simulink model "neural_30102019"  (R2018b)
settings: Solver=VariableStepAuto  StartTime=0.0  StopTime=10.0  RelTol=1e-3
libraries: neural x206
(part 4 of 5)

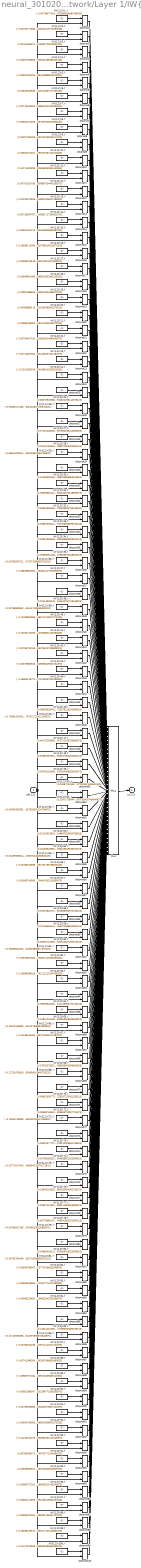
== system neural_30102019/NARX Neural Network/Layer 1/IW{1,2} ==
  "pd{1,2}" : Inport  PortDimensions=10  SampleTime=1
      mask Display: e = 0.06;c1 = [120 230 180]/255;c2 = ([120 230 180]+0)/(256+128);c3 = ([120 230 180]+128)/(256+128);patch([0 1 1 0],[0 0 1 1],c1);patch([0 1 1 1-e 1-e 0+e],[0 0 1 1-e 0+e 0+e],c2);patch([0 0 1 1-e 0+e 0+e],[0 1 1 1-e 1-e 0+e],c3);plot([0 1 1 0 0],[0 0 1 1 0]);
  "IW{1,2}(1,:)'" : Constant  Value=[-0.00798677624919284789850593142546131275594234466552734375;-0.07503946903610680951857148102135397493839263916015625;0.06674643641486444067822958459146320819854736328125;0.049874328743752534276456600537130725570023059844970703125;0.0265489642087564405026345326632508658803999423980712890625;0.013581459089883285429323223070241510868072509765625;0.0285023478571909405498985279336920939385890960693359375;-0.0283260124732715896922474740904362988658249378204345703125;-0.0021890880565128534827878947766066630720160901546478271484375;-0.0190405198631498108474691122182775870896875858306884765625]
      mask Display: e = 0.06;c1 = [120 150 230]/255;c2 = ([120 150 230]+0)/383;c3 = ([120 150 230]+128)/383;patch([0 1 1 0],[0 0 1 1],c1);patch([0 1 1 1-e 1-e 0+e],[0 0 1 1-e 0+e 0+e],c2);patch([0 0 1 1-e 0+e 0+e],[0 1 1 1-e 1-e 0+e],c3);plot([0 1 1 0 0],[0 0 1 1 0]);disp('Weights');
  "IW{1,2}(10,:)'" : Constant  Value=[0.006046723010521692399932280892471680999733507633209228515625;0.061987225392220464403880697545901057310402393341064453125;-0.05670670786149811792853370207012630999088287353515625;-0.04254940000158814739084078837549895979464054107666015625;-0.0229325631839031769676484628917023655958473682403564453125;-0.0119859294762603429962410928055760450661182403564453125;-0.024522060071650482460103859239097801037132740020751953125;0.0229149815121166035292166185399764799512922763824462890625;0.0011335620226404640072115359572535453480668365955352783203125;0.01529158681787430064391575257332078763283789157867431640625]
      mask Display: e = 0.06;c1 = [120 150 230]/255;c2 = ([120 150 230]+0)/383;c3 = ([120 150 230]+128)/383;patch([0 1 1 0],[0 0 1 1],c1);patch([0 1 1 1-e 1-e 0+e],[0 0 1 1-e 0+e 0+e],c2);patch([0 0 1 1-e 0+e 0+e],[0 1 1 1-e 1-e 0+e],c3);plot([0 1 1 0 0],[0 0 1 1 0]);disp('Weights');
  "IW{1,2}(100,:)'" : Constant  Value=[-0.2141767990978555580294795390727813355624675750732421875;-0.128247192817492250416222532294341363012790679931640625;-0.396524834829238503886017497279681265354156494140625;0.3360193962545301449296175633207894861698150634765625;-0.14726526146259144578465338781825266778469085693359375;0.259370633440820841375540339868166483938694000244140625;-0.0037662832053176639561520300247821069206111133098602294921875;0.213933770737092021629877081068116240203380584716796875;0.1274296387092574978083803216577507555484771728515625;0.1001974994320343481657431539133540354669094085693359375]
      mask Display: e = 0.06;c1 = [120 150 230]/255;c2 = ([120 150 230]+0)/383;c3 = ([120 150 230]+128)/383;patch([0 1 1 0],[0 0 1 1],c1);patch([0 1 1 1-e 1-e 0+e],[0 0 1 1-e 0+e 0+e],c2);patch([0 0 1 1-e 0+e 0+e],[0 1 1 1-e 1-e 0+e],c3);plot([0 1 1 0 0],[0 0 1 1 0]);disp('Weights');
  "IW{1,2}(11,:)'" : Constant  Value=[0.421713282934833733062163219074136577546596527099609375;-0.259807602882639099295403184441966004669666290283203125;-0.27575785944389252790642785839736461639404296875;-0.507622809805222008350256146513856947422027587890625;-0.366517809471706257351542035394231788814067840576171875;-0.31407420620104453679033440494094975292682647705078125;-0.27804590867977185819626129159587435424327850341796875;0.1700226487380198381327289780529099516570568084716796875;0.01439665602552794680668579729854172910563647747039794921875;-0.29063000749984058135311215664842166006565093994140625]
      mask Display: e = 0.06;c1 = [120 150 230]/255;c2 = ([120 150 230]+0)/383;c3 = ([120 150 230]+128)/383;patch([0 1 1 0],[0 0 1 1],c1);patch([0 1 1 1-e 1-e 0+e],[0 0 1 1-e 0+e 0+e],c2);patch([0 0 1 1-e 0+e 0+e],[0 1 1 1-e 1-e 0+e],c3);plot([0 1 1 0 0],[0 0 1 1 0]);disp('Weights');
  "IW{1,2}(12,:)'" : Constant  Value=[0.007616107951092995591302337032857394660823047161102294921875;0.072611082900980505883126170374453067779541015625;-0.0648315312200906379569431692289072088897228240966796875;-0.048465470835274519767477130471888813190162181854248046875;-0.025819065849659532385640403617799165658652782440185546875;-0.01322418345371845736779814473038641153834760189056396484375;-0.027704240289464894531068495098224957473576068878173828125;0.0273498164796031305312506987093001953326165676116943359375;0.002044885299220683579080048986043038894422352313995361328125;0.0183814053611497628393234293753266683779656887054443359375]
      mask Display: e = 0.06;c1 = [120 150 230]/255;c2 = ([120 150 230]+0)/383;c3 = ([120 150 230]+128)/383;patch([0 1 1 0],[0 0 1 1],c1);patch([0 1 1 1-e 1-e 0+e],[0 0 1 1-e 0+e 0+e],c2);patch([0 0 1 1-e 0+e 0+e],[0 1 1 1-e 1-e 0+e],c3);plot([0 1 1 0 0],[0 0 1 1 0]);disp('Weights');
  "IW{1,2}(13,:)'" : Constant  Value=[-0.0010537055901131326708652924395437366911210119724273681640625;-0.0239240992321591468272590219612538930959999561309814453125;0.0255710545558940662014268951907070004381239414215087890625;0.0194741137923734007608711493730879737995564937591552734375;0.01128805501537038895321085618661527405492961406707763671875;0.006558522094036949023898586119685205630958080291748046875;0.01174088385979915084844638073491296381689608097076416015625;-0.0077679497450684475978732734802179038524627685546875;0.0011445875772253988507387578721363752265460789203643798828125;-0.004942996574598020921575969310879372642375528812408447265625]
      mask Display: e = 0.06;c1 = [120 150 230]/255;c2 = ([120 150 230]+0)/383;c3 = ([120 150 230]+128)/383;patch([0 1 1 0],[0 0 1 1],c1);patch([0 1 1 1-e 1-e 0+e],[0 0 1 1-e 0+e 0+e],c2);patch([0 0 1 1-e 0+e 0+e],[0 1 1 1-e 1-e 0+e],c3);plot([0 1 1 0 0],[0 0 1 1 0]);disp('Weights');
  "IW{1,2}(14,:)'" : Constant  Value=[0.007355647677175658309678407675846756319515407085418701171875;0.07087343205888226027600040879406151361763477325439453125;-0.0634921597831986928017755644759745337069034576416015625;-0.0474884902285650500886049485416151583194732666015625;-0.025332830322819466228878582114703021943569183349609375;-0.01300591691238471743485849430044254404492676258087158203125;-0.0271698679463006353973497652987134642899036407470703125;0.026631749153002683139224160413505160249769687652587890625;0.00190872735472459066630168678102563717402517795562744140625;0.01788489226589433378489246706521953456103801727294921875]
      mask Display: e = 0.06;c1 = [120 150 230]/255;c2 = ([120 150 230]+0)/383;c3 = ([120 150 230]+128)/383;patch([0 1 1 0],[0 0 1 1],c1);patch([0 1 1 1-e 1-e 0+e],[0 0 1 1-e 0+e 0+e],c2);patch([0 0 1 1-e 0+e 0+e],[0 1 1 1-e 1-e 0+e],c3);plot([0 1 1 0 0],[0 0 1 1 0]);disp('Weights');
  "IW{1,2}(15,:)'" : Constant  Value=[-0.00814161173255857802122381627896174904890358448028564453125;-0.075994613132684296630259268567897379398345947265625;0.06753453343498776184627985230690683238208293914794921875;0.05046449069054280422985669929403229616582393646240234375;0.0268793826447808713309139960756510845385491847991943359375;0.013766439113115279402332902236594236455857753753662109375;0.0288593792420822337074781671617529354989528656005859375;-0.028685856450662162997478077386404038406908512115478515625;-0.0022058677687657114903363453350948475417681038379669189453125;-0.01926966050066114544137008124380372464656829833984375]
      mask Display: e = 0.06;c1 = [120 150 230]/255;c2 = ([120 150 230]+0)/383;c3 = ([120 150 230]+128)/383;patch([0 1 1 0],[0 0 1 1],c1);patch([0 1 1 1-e 1-e 0+e],[0 0 1 1-e 0+e 0+e],c2);patch([0 0 1 1-e 0+e 0+e],[0 1 1 1-e 1-e 0+e],c3);plot([0 1 1 0 0],[0 0 1 1 0]);disp('Weights');
  "IW{1,2}(16,:)'" : Constant  Value=[-0.29668115008275630639644759867223910987377166748046875;-0.1429409359042553562257893418063758872449398040771484375;-0.003996746244826050731280275840617832727730274200439453125;0.1368595726162756542887422028798027895390987396240234375;-0.133843639625026378237038215956999920308589935302734375;-0.382580478673099577680005722868372686207294464111328125;-0.63959980856266540616417159981210716068744659423828125;-0.0904466078387958505313548585036187432706356048583984375;-0.01188476076923118858463812586023777839727699756622314453125;0.421520946410732733067305844087968580424785614013671875]
      mask Display: e = 0.06;c1 = [120 150 230]/255;c2 = ([120 150 230]+0)/383;c3 = ([120 150 230]+128)/383;patch([0 1 1 0],[0 0 1 1],c1);patch([0 1 1 1-e 1-e 0+e],[0 0 1 1-e 0+e 0+e],c2);patch([0 0 1 1-e 0+e 0+e],[0 1 1 1-e 1-e 0+e],c3);plot([0 1 1 0 0],[0 0 1 1 0]);disp('Weights');
  "IW{1,2}(17,:)'" : Constant  Value=[-0.0089611951806888960614383421443562838248908519744873046875;-0.080259490925016996332175267525599338114261627197265625;0.0713183404309283008881692467184620909392833709716796875;0.05343656199492992364685761685905163176357746124267578125;0.02883618272078312949613376758861704729497432708740234375;0.01506443241417236567070148112179595045745372772216796875;0.030848081919005641837738806998459040187299251556396484375;-0.0300637610862332128880414217064753756858408451080322265625;-0.00187828771485964540581548032349701315979473292827606201171875;-0.0199686849717214086330496769505771226249635219573974609375]
      mask Display: e = 0.06;c1 = [120 150 230]/255;c2 = ([120 150 230]+0)/383;c3 = ([120 150 230]+128)/383;patch([0 1 1 0],[0 0 1 1],c1);patch([0 1 1 1-e 1-e 0+e],[0 0 1 1-e 0+e 0+e],c2);patch([0 0 1 1-e 0+e 0+e],[0 1 1 1-e 1-e 0+e],c3);plot([0 1 1 0 0],[0 0 1 1 0]);disp('Weights');
  "IW{1,2}(18,:)'" : Constant  Value=[0.00848961486607587891006776459335014806129038333892822265625;0.07767125028041090006869495709906914271414279937744140625;-0.0690349437182005976065823915632790885865688323974609375;-0.051627200903625637684601912269499734975397586822509765625;-0.0276423307452806042705528710712314932607114315032958984375;-0.0142761761840401735224048707095789723098278045654296875;-0.0296519928027474018172870984244582359679043292999267578125;0.029209814683932501522267699556323350407183170318603515625;0.00206227852408806359985060652206811937503516674041748046875;0.0195439959360052158132692312619838048703968524932861328125]
      mask Display: e = 0.06;c1 = [120 150 230]/255;c2 = ([120 150 230]+0)/383;c3 = ([120 150 230]+128)/383;patch([0 1 1 0],[0 0 1 1],c1);patch([0 1 1 1-e 1-e 0+e],[0 0 1 1-e 0+e 0+e],c2);patch([0 0 1 1-e 0+e 0+e],[0 1 1 1-e 1-e 0+e],c3);plot([0 1 1 0 0],[0 0 1 1 0]);disp('Weights');
  "IW{1,2}(19,:)'" : Constant  Value=[0.0085796862633227659322709968137132818810641765594482421875;0.07930105914873393502251275322123547084629535675048828125;-0.0701868817899373442781296716930228285491466522216796875;-0.0524578341906625500445926491011050529778003692626953125;-0.0279347662272163045626971467072507948614656925201416015625;-0.01430608406650272536320134264542502933181822299957275390625;-0.02998821634027049043424995034001767635345458984375;0.0300247568622749316791242790714022703468799591064453125;0.0023842574512983236677265974634565282030962407588958740234375;0.0201306524346432751115809622888264129869639873504638671875]
      mask Display: e = 0.06;c1 = [120 150 230]/255;c2 = ([120 150 230]+0)/383;c3 = ([120 150 230]+128)/383;patch([0 1 1 0],[0 0 1 1],c1);patch([0 1 1 1-e 1-e 0+e],[0 0 1 1-e 0+e 0+e],c2);patch([0 0 1 1-e 0+e 0+e],[0 1 1 1-e 1-e 0+e],c3);plot([0 1 1 0 0],[0 0 1 1 0]);disp('Weights');
  "IW{1,2}(2,:)'" : Constant  Value=[-0.007357745885256144167951841694730319431982934474945068359375;-0.070887480606621477985385126885375939309597015380859375;0.063502940384915607108240465095150284469127655029296875;0.04749634226454813035189772563171572983264923095703125;0.0253367055119268387575193202110312995500862598419189453125;0.01300762238957645956782815943597597652114927768707275390625;0.0271741310243342193420090779909514822065830230712890625;-0.02663758450105276065489334769154083915054798126220703125;-0.001909879321627074542921942423845393932424485683441162109375;-0.01788894417836141281785700130058103241026401519775390625]
      mask Display: e = 0.06;c1 = [120 150 230]/255;c2 = ([120 150 230]+0)/383;c3 = ([120 150 230]+128)/383;patch([0 1 1 0],[0 0 1 1],c1);patch([0 1 1 1-e 1-e 0+e],[0 0 1 1-e 0+e 0+e],c2);patch([0 0 1 1-e 0+e 0+e],[0 1 1 1-e 1-e 0+e],c3);plot([0 1 1 0 0],[0 0 1 1 0]);disp('Weights');
  "IW{1,2}(20,:)'" : Constant  Value=[0.00486889115257779607481847250483042444102466106414794921875;0.053814783214718685255828489744089893065392971038818359375;-0.05040437383040684282686783035387634299695491790771484375;-0.037941123090531068962061311822253628633916378021240234375;-0.0206956196985309155700338834549256716854870319366455078125;-0.01103117006039725823962616146900472813285887241363525390625;-0.02204589041565323259685982293376582674682140350341796875;0.01952046424261948132095056962498347274959087371826171875;0.0004479422599597729479255214801725060169701464474201202392578125;0.012932389808863638258618067311545019038021564483642578125]
      mask Display: e = 0.06;c1 = [120 150 230]/255;c2 = ([120 150 230]+0)/383;c3 = ([120 150 230]+128)/383;patch([0 1 1 0],[0 0 1 1],c1);patch([0 1 1 1-e 1-e 0+e],[0 0 1 1-e 0+e 0+e],c2);patch([0 0 1 1-e 0+e 0+e],[0 1 1 1-e 1-e 0+e],c3);plot([0 1 1 0 0],[0 0 1 1 0]);disp('Weights');
  "IW{1,2}(21,:)'" : Constant  Value=[0.00866763351667522441434954316719085909426212310791015625;0.0782513990823368865701326058115228079259395599365234375;-0.06959131286961850459960032821982167661190032958984375;-0.052074545671010115388543937342546996660530567169189453125;-0.0279930318366197854185184468178704264573752880096435546875;-0.0145387189400555984220009264618056477047502994537353515625;-0.0299946157684723470338017392577967257238924503326416015625;0.0293345517321344957661910513024849933572113513946533203125;0.0019256041878866268605985379025469228508882224559783935546875;0.01957585198270024584576987081163679249584674835205078125]
      mask Display: e = 0.06;c1 = [120 150 230]/255;c2 = ([120 150 230]+0)/383;c3 = ([120 150 230]+128)/383;patch([0 1 1 0],[0 0 1 1],c1);patch([0 1 1 1-e 1-e 0+e],[0 0 1 1-e 0+e 0+e],c2);patch([0 0 1 1-e 0+e 0+e],[0 1 1 1-e 1-e 0+e],c3);plot([0 1 1 0 0],[0 0 1 1 0]);disp('Weights');
  "IW{1,2}(22,:)'" : Constant  Value=[-0.00708497015945106119183538595507343416102230548858642578125;-0.06905513385735366493900500017844024114310741424560546875;0.062100633166464781764748437353773624636232852935791015625;0.046475737701175169613865278961384319700300693511962890625;0.024835895369398175436259634807356633245944976806640625;0.0127901955732843443380719605784179293550550937652587890625;0.026622792341062316567867895855670212768018245697021484375;-0.0258740150793133893980524362632422707974910736083984375;-0.00175537877912571547989184495008885278366506099700927734375;-0.0173574384835007526628469776142082992009818553924560546875]
      mask Display: e = 0.06;c1 = [120 150 230]/255;c2 = ([120 150 230]+0)/383;c3 = ([120 150 230]+128)/383;patch([0 1 1 0],[0 0 1 1],c1);patch([0 1 1 1-e 1-e 0+e],[0 0 1 1-e 0+e 0+e],c2);patch([0 0 1 1-e 0+e 0+e],[0 1 1 1-e 1-e 0+e],c3);plot([0 1 1 0 0],[0 0 1 1 0]);disp('Weights');
  "IW{1,2}(23,:)'" : Constant  Value=[-0.0074483790066924328299169388856171281076967716217041015625;-0.07149358462194989327631589048905880190432071685791015625;0.06396867056060819012319740295424708165228366851806640625;0.0478356987540748679332835990862804464995861053466796875;0.025504621020149088883588461840190575458109378814697265625;0.01308197665947793790486297638153700972907245159149169921875;0.027358797069702144033609414464081055484712123870849609375;-0.0268889540057255758964682712530702701769769191741943359375;-0.0019589140339770125774643272364983204170130193233489990234375;-0.0180632731988428739400287525995736359618604183197021484375]
      mask Display: e = 0.06;c1 = [120 150 230]/255;c2 = ([120 150 230]+0)/383;c3 = ([120 150 230]+128)/383;patch([0 1 1 0],[0 0 1 1],c1);patch([0 1 1 1-e 1-e 0+e],[0 0 1 1-e 0+e 0+e],c2);patch([0 0 1 1-e 0+e 0+e],[0 1 1 1-e 1-e 0+e],c3);plot([0 1 1 0 0],[0 0 1 1 0]);disp('Weights');
  "IW{1,2}(24,:)'" : Constant  Value=[-0.21911639010605588051561198881245218217372894287109375;-0.01243976575982347516913240070834945072419941425323486328125;-0.276747236623042791592297362512908875942230224609375;0.331513151846347275952808786314562894403934478759765625;0.01530829276420064312402846695704283774830400943756103515625;-0.438908061994073506184577126987278461456298828125;-0.256665691825826047800518381336587481200695037841796875;0.1502781112545034936101018274712259881198406219482421875;-0.060289536450497317743302261305871070362627506256103515625;0.43710829934427819498665712671936489641666412353515625]
      mask Display: e = 0.06;c1 = [120 150 230]/255;c2 = ([120 150 230]+0)/383;c3 = ([120 150 230]+128)/383;patch([0 1 1 0],[0 0 1 1],c1);patch([0 1 1 1-e 1-e 0+e],[0 0 1 1-e 0+e 0+e],c2);patch([0 0 1 1-e 0+e 0+e],[0 1 1 1-e 1-e 0+e],c3);plot([0 1 1 0 0],[0 0 1 1 0]);disp('Weights');
  "IW{1,2}(25,:)'" : Constant  Value=[0.6057391656667754364917755083297379314899444580078125;0.254106170497063021951333894321578554809093475341796875;-0.265690881170252690690603003531577996909618377685546875;-0.429186757129940088528741171103320084512233734130859375;-0.3187917527291614927520413402817212045192718505859375;0.0969355372234030621125810966987046413123607635498046875;-0.282662417338566618330020219218567945063114166259765625;0.13774202595325746312227011003415100276470184326171875;-0.0314014927503679375231371295740245841443538665771484375;-0.155522626980701517140914802439510822296142578125]
      mask Display: e = 0.06;c1 = [120 150 230]/255;c2 = ([120 150 230]+0)/383;c3 = ([120 150 230]+128)/383;patch([0 1 1 0],[0 0 1 1],c1);patch([0 1 1 1-e 1-e 0+e],[0 0 1 1-e 0+e 0+e],c2);patch([0 0 1 1-e 0+e 0+e],[0 1 1 1-e 1-e 0+e],c3);plot([0 1 1 0 0],[0 0 1 1 0]);disp('Weights');
  "IW{1,2}(26,:)'" : Constant  Value=[-0.006801714662381373212307611453297795378603041172027587890625;-0.06714051525852171575792226576595567166805267333984375;0.06063991378496670636710774715538718737661838531494140625;0.045413235239481146432449776284556719474494457244873046875;0.024318707141640506785851272297804825939238071441650390625;0.01256986612047581060302992028709923033602535724639892578125;0.026052733747598109947940514530273503623902797698974609375;-0.0250729610539233427335403803226654417812824249267578125;-0.00158832976997171364426375550493730770540423691272735595703125;-0.0167982994126852532013050023351752315647900104522705078125]
      mask Display: e = 0.06;c1 = [120 150 230]/255;c2 = ([120 150 230]+0)/383;c3 = ([120 150 230]+128)/383;patch([0 1 1 0],[0 0 1 1],c1);patch([0 1 1 1-e 1-e 0+e],[0 0 1 1-e 0+e 0+e],c2);patch([0 0 1 1-e 0+e 0+e],[0 1 1 1-e 1-e 0+e],c3);plot([0 1 1 0 0],[0 0 1 1 0]);disp('Weights');
  "IW{1,2}(27,:)'" : Constant  Value=[0.07131128009140497159279448169399984180927276611328125;-0.0021649104732030465501890770241288919351063668727874755859375;0.357824589089750066950301743418094702064990997314453125;0.085457057636947830747686793984030373394489288330078125;0.2253782000391293116603463886349345557391643524169921875;-0.1387275976291638956983121033772476948797702789306640625;-0.1631566888323170705366038646388915367424488067626953125;-0.01104966204846205383993673621034758980385959148406982421875;0.1563081036359025011162060536662465892732143402099609375;0.27629181597915997148362521329545415937900543212890625]
      mask Display: e = 0.06;c1 = [120 150 230]/255;c2 = ([120 150 230]+0)/383;c3 = ([120 150 230]+128)/383;patch([0 1 1 0],[0 0 1 1],c1);patch([0 1 1 1-e 1-e 0+e],[0 0 1 1-e 0+e 0+e],c2);patch([0 0 1 1-e 0+e 0+e],[0 1 1 1-e 1-e 0+e],c3);plot([0 1 1 0 0],[0 0 1 1 0]);disp('Weights');
  "IW{1,2}(28,:)'" : Constant  Value=[0.10542750616784980766116319728098460473120212554931640625;0.00983497914079346606530673824408950167708098888397216796875;0.1352709594469807818928330789276515133678913116455078125;0.419651828406918558922455986248678527772426605224609375;-0.255329452737788453742240335486712865531444549560546875;-0.286151047620699150453305037444806657731533050537109375;0.23033272063401721840847358180326409637928009033203125;0.13463854237295047600042607882642187178134918212890625;0.079277104628094618998801479392568580806255340576171875;-0.13570287260015423402848000478115864098072052001953125]
      mask Display: e = 0.06;c1 = [120 150 230]/255;c2 = ([120 150 230]+0)/383;c3 = ([120 150 230]+128)/383;patch([0 1 1 0],[0 0 1 1],c1);patch([0 1 1 1-e 1-e 0+e],[0 0 1 1-e 0+e 0+e],c2);patch([0 0 1 1-e 0+e 0+e],[0 1 1 1-e 1-e 0+e],c3);plot([0 1 1 0 0],[0 0 1 1 0]);disp('Weights');
  "IW{1,2}(29,:)'" : Constant  Value=[-0.56624376541417753561091785741155035793781280517578125;0.24101456158054113121380623852019198238849639892578125;0.110371363230960917167777779468451626598834991455078125;0.116837946971778905425054517763783223927021026611328125;0.0032340983457502451951792732387502837809734046459197998046875;-0.08506937579697225471075938685316941700875759124755859375;-0.016568341644388896727324578250772901810705661773681640625;0.417247058757125810490862249935162253677845001220703125;0.4221235175928590432903320106561295688152313232421875;-0.046730484977605825369639802602250711061060428619384765625]
      mask Display: e = 0.06;c1 = [120 150 230]/255;c2 = ([120 150 230]+0)/383;c3 = ([120 150 230]+128)/383;patch([0 1 1 0],[0 0 1 1],c1);patch([0 1 1 1-e 1-e 0+e],[0 0 1 1-e 0+e 0+e],c2);patch([0 0 1 1-e 0+e 0+e],[0 1 1 1-e 1-e 0+e],c3);plot([0 1 1 0 0],[0 0 1 1 0]);disp('Weights');
  "IW{1,2}(3,:)'" : Constant  Value=[0.007534909710501822531492077672510276897810399532318115234375;0.07207083989842300031369859425467438995838165283203125;-0.0644135831885673526553404144578962586820125579833984375;-0.048160216158633979699477123403994482941925525665283203125;-0.025666118012424542216276535100405453704297542572021484375;-0.01315445687860261440860210058190205018036067485809326171875;-0.0275362839360003795741160814714021398685872554779052734375;0.027127517144081396416321894093925948254764080047607421875;0.0020041753028468820875540590265018181526102125644683837890625;0.0182282436409296096091470218425456550903618335723876953125]
      mask Display: e = 0.06;c1 = [120 150 230]/255;c2 = ([120 150 230]+0)/383;c3 = ([120 150 230]+128)/383;patch([0 1 1 0],[0 0 1 1],c1);patch([0 1 1 1-e 1-e 0+e],[0 0 1 1-e 0+e 0+e],c2);patch([0 0 1 1-e 0+e 0+e],[0 1 1 1-e 1-e 0+e],c3);plot([0 1 1 0 0],[0 0 1 1 0]);disp('Weights');
  "IW{1,2}(30,:)'" : Constant  Value=[0.242959481634212604017619696605834178626537322998046875;-0.0417741403241910502774913993562222458422183990478515625;0.658235812223002536569538278854452073574066162109375;-0.33141388019204198744915856877923943102359771728515625;0.416733972177876166309573591206572018563747406005859375;-0.085797801298780840273394687756081111729145050048828125;-0.1883367268382012127414526503343950025737285614013671875;0.09436084962322231761699953267452656291425228118896484375;0.1777182592148270068310722535898094065487384796142578125;0.366611824067617053657386350096203386783599853515625]
      mask Display: e = 0.06;c1 = [120 150 230]/255;c2 = ([120 150 230]+0)/383;c3 = ([120 150 230]+128)/383;patch([0 1 1 0],[0 0 1 1],c1);patch([0 1 1 1-e 1-e 0+e],[0 0 1 1-e 0+e 0+e],c2);patch([0 0 1 1-e 0+e 0+e],[0 1 1 1-e 1-e 0+e],c3);plot([0 1 1 0 0],[0 0 1 1 0]);disp('Weights');
  "IW{1,2}(31,:)'" : Constant  Value=[0.00839862424112747772697584736079079448245465755462646484375;0.07731160948217614958810628422725130803883075714111328125;-0.06869771665354824918825471513628144748508930206298828125;-0.051360203720061357868242879476383677683770656585693359375;-0.02744912374357481865683183741566608659923076629638671875;-0.01413725550662080741870507694102343521080911159515380859375;-0.02945715178367015740779066845789202488958835601806640625;0.0291156286548447003348361050711901043541729450225830078125;0.002121742504950652717654602241736938594840466976165771484375;0.01950610736164447300833302278988412581384181976318359375]
      mask Display: e = 0.06;c1 = [120 150 230]/255;c2 = ([120 150 230]+0)/383;c3 = ([120 150 230]+128)/383;patch([0 1 1 0],[0 0 1 1],c1);patch([0 1 1 1-e 1-e 0+e],[0 0 1 1-e 0+e 0+e],c2);patch([0 0 1 1-e 0+e 0+e],[0 1 1 1-e 1-e 0+e],c3);plot([0 1 1 0 0],[0 0 1 1 0]);disp('Weights');
  "IW{1,2}(32,:)'" : Constant  Value=[0.369346364835059171038977865464403294026851654052734375;0.09681434486543329109853317504530423320829868316650390625;0.582344035522904146517930712434463202953338623046875;-0.56086275654786998945411369277280755341053009033203125;0.039131820943061980389021670134752639569342136383056640625;-0.386360337036403489463509686174802482128143310546875;-0.2685299897506923105794385264744050800800323486328125;-0.1252979787581995907430609804578125476837158203125;0.0768068550977881459029816824113368056714534759521484375;0.354604923895247614584746997934416867792606353759765625]
      mask Display: e = 0.06;c1 = [120 150 230]/255;c2 = ([120 150 230]+0)/383;c3 = ([120 150 230]+128)/383;patch([0 1 1 0],[0 0 1 1],c1);patch([0 1 1 1-e 1-e 0+e],[0 0 1 1-e 0+e 0+e],c2);patch([0 0 1 1-e 0+e 0+e],[0 1 1 1-e 1-e 0+e],c3);plot([0 1 1 0 0],[0 0 1 1 0]);disp('Weights');
  "IW{1,2}(33,:)'" : Constant  Value=[0.0085303821461721988927973114869018900208175182342529296875;0.0792581604486289059696701997381751425564289093017578125;-0.07003614384118529712086598237874568440020084381103515625;-0.052315847801904492853086736658951849676668643951416015625;-0.0277763320123694014418536113453228608705103397369384765625;-0.0141483117667682879725621347688502282835543155670166015625;-0.0298255084064666942111898606526665389537811279296875;0.030092315734682129058086275108507834374904632568359375;0.0025184814520494663674099466987854611943475902080535888671875;0.0202188966654386244325980470648573827929794788360595703125]
      mask Display: e = 0.06;c1 = [120 150 230]/255;c2 = ([120 150 230]+0)/383;c3 = ([120 150 230]+128)/383;patch([0 1 1 0],[0 0 1 1],c1);patch([0 1 1 1-e 1-e 0+e],[0 0 1 1-e 0+e 0+e],c2);patch([0 0 1 1-e 0+e 0+e],[0 1 1 1-e 1-e 0+e],c3);plot([0 1 1 0 0],[0 0 1 1 0]);disp('Weights');
  "IW{1,2}(34,:)'" : Constant  Value=[0.20867893848387997213222888603922910988330841064453125;0.2143074769810318913609847868428914807736873626708984375;-0.24355015505442023648896565646282397210597991943359375;-0.132314619513283882046295047985040582716464996337890625;-0.1363921224583313496214742599477176554501056671142578125;-0.03469070119655058570540262508075102232396602630615234375;0.01404042959988481033273277631678865873254835605621337890625;-0.04500329280021771183317724762673606164753437042236328125;-0.0592947686487854397352492696882109157741069793701171875;-0.0259059849739228138798541323239987832494080066680908203125]
      mask Display: e = 0.06;c1 = [120 150 230]/255;c2 = ([120 150 230]+0)/383;c3 = ([120 150 230]+128)/383;patch([0 1 1 0],[0 0 1 1],c1);patch([0 1 1 1-e 1-e 0+e],[0 0 1 1-e 0+e 0+e],c2);patch([0 0 1 1-e 0+e 0+e],[0 1 1 1-e 1-e 0+e],c3);plot([0 1 1 0 0],[0 0 1 1 0]);disp('Weights');
  "IW{1,2}(35,:)'" : Constant  Value=[0.00960661436772869241351724411970280925743281841278076171875;-0.22744418547777522920938508832477964460849761962890625;0.1376400625764244434190430865783127956092357635498046875;0.049973371980813967307977208065494778566062450408935546875;0.53630542600377995032800981789478100836277008056640625;0.133657341437658505611807413515634834766387939453125;-0.0175443175098067942474511227146649616770446300506591796875;-0.139895193403781537000440948759205639362335205078125;-0.22148819212720349813849907150142826139926910400390625;-0.34148234936702082098491928263683803379535675048828125]
      mask Display: e = 0.06;c1 = [120 150 230]/255;c2 = ([120 150 230]+0)/383;c3 = ([120 150 230]+128)/383;patch([0 1 1 0],[0 0 1 1],c1);patch([0 1 1 1-e 1-e 0+e],[0 0 1 1-e 0+e 0+e],c2);patch([0 0 1 1-e 0+e 0+e],[0 1 1 1-e 1-e 0+e],c3);plot([0 1 1 0 0],[0 0 1 1 0]);disp('Weights');
  "IW{1,2}(36,:)'" : Constant  Value=[-0.007635870215056389694041616422737206448800861835479736328125;-0.072742325179648570365742443755152635276317596435546875;0.064933342151428707911264837093767710030078887939453125;0.04853990443110346719723935393631109036505222320556640625;0.0258565423170550034992487553608953021466732025146484375;0.0132414566793657741128331650770633132196962833404541015625;0.0277453705097093945852737562063339282758533954620361328125;-0.027403647958128544981359908661033841781318187713623046875;-0.002054482437872061362238440551664098165929317474365234375;-0.0184183932665478063139818942772762966342270374298095703125]
      mask Display: e = 0.06;c1 = [120 150 230]/255;c2 = ([120 150 230]+0)/383;c3 = ([120 150 230]+128)/383;patch([0 1 1 0],[0 0 1 1],c1);patch([0 1 1 1-e 1-e 0+e],[0 0 1 1-e 0+e 0+e],c2);patch([0 0 1 1-e 0+e 0+e],[0 1 1 1-e 1-e 0+e],c3);plot([0 1 1 0 0],[0 0 1 1 0]);disp('Weights');
  "IW{1,2}(37,:)'" : Constant  Value=[-0.388498550637164152821156903883093036711215972900390625;0.49736943056161198040143744947272352874279022216796875;0.478056688340715962848292974740616045892238616943359375;-0.187262534023833915330925492526148445904254913330078125;-0.5586836521030094093731577231665141880512237548828125;-0.2406663885132401536903756777974194847047328948974609375;-0.084619108831960276884132099439739249646663665771484375;-0.050153435080850440608291052058120840229094028472900390625;0.19755419481900471367907812236808240413665771484375;0.3355238901682671137649549564230255782604217529296875]
      mask Display: e = 0.06;c1 = [120 150 230]/255;c2 = ([120 150 230]+0)/383;c3 = ([120 150 230]+128)/383;patch([0 1 1 0],[0 0 1 1],c1);patch([0 1 1 1-e 1-e 0+e],[0 0 1 1-e 0+e 0+e],c2);patch([0 0 1 1-e 0+e 0+e],[0 1 1 1-e 1-e 0+e],c3);plot([0 1 1 0 0],[0 0 1 1 0]);disp('Weights');
  "IW{1,2}(38,:)'" : Constant  Value=[0.2511490324976339838514149960246868431568145751953125;-0.128348381365441521761994181360932998359203338623046875;0.06819919537138234566508998568679089657962322235107421875;0.12749848841446420610878931256593205034732818603515625;0.363153841185997972029753100287052802741527557373046875;-0.1776700490802503029641457032994367182254791259765625;-0.242976706441258072377564758426160551607608795166015625;0.06730211923017988262518684905444388277828693389892578125;0.044546208769704047358839460457602399401366710662841796875;-0.061490912827307557531053561206135782413184642791748046875]
      mask Display: e = 0.06;c1 = [120 150 230]/255;c2 = ([120 150 230]+0)/383;c3 = ([120 150 230]+128)/383;patch([0 1 1 0],[0 0 1 1],c1);patch([0 1 1 1-e 1-e 0+e],[0 0 1 1-e 0+e 0+e],c2);patch([0 0 1 1-e 0+e 0+e],[0 1 1 1-e 1-e 0+e],c3);plot([0 1 1 0 0],[0 0 1 1 0]);disp('Weights');
  "IW{1,2}(39,:)'" : Constant  Value=[-0.007688396320664891460394674282952109933830797672271728515625;-0.0730906087948191285352805834918399341404438018798828125;0.0652041463789563013886407816244172863662242889404296875;0.048738059175677757306477388965504360385239124298095703125;0.025956715087612984571574514802705380134284496307373046875;0.01328804358375379988943532083567333756946027278900146484375;0.0278552561390369157745539041570737026631832122802734375;-0.027546115541961457839903459898778237402439117431640625;-0.00207929379404799864750064131158069358207285404205322265625;-0.018516053770908987019527813799868454225361347198486328125]
      mask Display: e = 0.06;c1 = [120 150 230]/255;c2 = ([120 150 230]+0)/383;c3 = ([120 150 230]+128)/383;patch([0 1 1 0],[0 0 1 1],c1);patch([0 1 1 1-e 1-e 0+e],[0 0 1 1-e 0+e 0+e],c2);patch([0 0 1 1-e 0+e 0+e],[0 1 1 1-e 1-e 0+e],c3);plot([0 1 1 0 0],[0 0 1 1 0]);disp('Weights');
  "IW{1,2}(4,:)'" : Constant  Value=[-0.00637465993407875138043738871829191339202225208282470703125;-0.06423379959766921387664950771068106405436992645263671875;0.058423277475708003392274036968956352211534976959228515625;0.04380010836220689374176373576119658537209033966064453125;0.0235373589926678346284649734343474847264587879180908203125;0.012240460689749967093664650974460528232157230377197265625;0.02519039216380007661921780481861787848174571990966796875;-0.0238551637414540496084924825481721200048923492431640625;-0.0013312815436777761073094961119522849912755191326141357421875;-0.0159477076986248751666597200937758316285908222198486328125]
      mask Display: e = 0.06;c1 = [120 150 230]/255;c2 = ([120 150 230]+0)/383;c3 = ([120 150 230]+128)/383;patch([0 1 1 0],[0 0 1 1],c1);patch([0 1 1 1-e 1-e 0+e],[0 0 1 1-e 0+e 0+e],c2);patch([0 0 1 1-e 0+e 0+e],[0 1 1 1-e 1-e 0+e],c3);plot([0 1 1 0 0],[0 0 1 1 0]);disp('Weights');
  "IW{1,2}(40,:)'" : Constant  Value=[-0.12408853983882535410021574762140517123043537139892578125;0.020518071422556787009039425129230949096381664276123046875;-0.86297703007523096641051552069257013499736785888671875;0.019005653693307235363452178944498882628977298736572265625;-0.3965235430061124777267878016573376953601837158203125;0.27873528930856605878574328016838990151882171630859375;0.0902666857515350695706501937820576131343841552734375;-0.33053230245538356424361836616299115121364593505859375;-0.256445713082278314853823530938825570046901702880859375;-0.344709948257618414846348287028376944363117218017578125]
      mask Display: e = 0.06;c1 = [120 150 230]/255;c2 = ([120 150 230]+0)/383;c3 = ([120 150 230]+128)/383;patch([0 1 1 0],[0 0 1 1],c1);patch([0 1 1 1-e 1-e 0+e],[0 0 1 1-e 0+e 0+e],c2);patch([0 0 1 1-e 0+e 0+e],[0 1 1 1-e 1-e 0+e],c3);plot([0 1 1 0 0],[0 0 1 1 0]);disp('Weights');
  "IW{1,2}(41,:)'" : Constant  Value=[-0.2302047629316530119591988068350474350154399871826171875;0.152307209577409896628097385473665781319141387939453125;0.464107114461969894048110063522472046315670013427734375;-0.09824756554074232095530305741704069077968597412109375;0.37441855927202472020809409514185972511768341064453125;0.174697502921786151919292251477600075304508209228515625;0.05809565230288650516943249613177613355219364166259765625;-0.131735813145984426153489721400546841323375701904296875;-0.1338508554063977118442352320926147513091564178466796875;-0.11075163766961894362683693771032267250120639801025390625]
      mask Display: e = 0.06;c1 = [120 150 230]/255;c2 = ([120 150 230]+0)/383;c3 = ([120 150 230]+128)/383;patch([0 1 1 0],[0 0 1 1],c1);patch([0 1 1 1-e 1-e 0+e],[0 0 1 1-e 0+e 0+e],c2);patch([0 0 1 1-e 0+e 0+e],[0 1 1 1-e 1-e 0+e],c3);plot([0 1 1 0 0],[0 0 1 1 0]);disp('Weights');
  "IW{1,2}(42,:)'" : Constant  Value=[-0.007667320498589581985460217339323207852430641651153564453125;-0.07295096307572047911182977486532763577997684478759765625;0.0650954509532313263520109103410504758358001708984375;0.048658492071152394109478933614809648133814334869384765625;0.0259164172440822966614337730106853996403515338897705078125;0.01326922610766675079962961802948484546504914760589599609375;0.0278110608413869135613349925506554427556693553924560546875;-0.02748906435609964338251387516720569692552089691162109375;-0.002069467152952960374567847878779502934776246547698974609375;-0.0184769882848117850127067640642053447663784027099609375]
      mask Display: e = 0.06;c1 = [120 150 230]/255;c2 = ([120 150 230]+0)/383;c3 = ([120 150 230]+128)/383;patch([0 1 1 0],[0 0 1 1],c1);patch([0 1 1 1-e 1-e 0+e],[0 0 1 1-e 0+e 0+e],c2);patch([0 0 1 1-e 0+e 0+e],[0 1 1 1-e 1-e 0+e],c3);plot([0 1 1 0 0],[0 0 1 1 0]);disp('Weights');
  "IW{1,2}(43,:)'" : Constant  Value=[-0.00876983503308761090655476522215394652448594570159912109375;-0.07983504610519187583150824139011092483997344970703125;0.07083189357068257752114703862389433197677135467529296875;0.053012995802292663116705995207667001523077487945556640625;0.028429550368470522803132638500756002031266689300537109375;0.0147229004691482867617224883360904641449451446533203125;0.03047162171117608064907500420304131694138050079345703125;-0.0300556306163373108952807655214201076887547969818115234375;-0.00211315403393556866529223725592601113021373748779296875;-0.0200475237310965247183869308855719282291829586029052734375]
      mask Display: e = 0.06;c1 = [120 150 230]/255;c2 = ([120 150 230]+0)/383;c3 = ([120 150 230]+128)/383;patch([0 1 1 0],[0 0 1 1],c1);patch([0 1 1 1-e 1-e 0+e],[0 0 1 1-e 0+e 0+e],c2);patch([0 0 1 1-e 0+e 0+e],[0 1 1 1-e 1-e 0+e],c3);plot([0 1 1 0 0],[0 0 1 1 0]);disp('Weights');
  "IW{1,2}(44,:)'" : Constant  Value=[-0.196831197211260355839357316654059104621410369873046875;0.004755009296519352619825315997559300740249454975128173828125;0.1973106764472241370089733436543610878288745880126953125;0.058391484374167475224215451135023613460361957550048828125;0.10999830257906619002117309946697787381708621978759765625;-0.29651652439407716332908648837474174797534942626953125;-0.0263660679632789739235132486783186323009431362152099609375;-0.00154190656894976295919474917894831378362141549587249755859375;-0.017058502831990986214893979422413394786417484283447265625;-0.181276988635208857747471711263642646372318267822265625]
      mask Display: e = 0.06;c1 = [120 150 230]/255;c2 = ([120 150 230]+0)/383;c3 = ([120 150 230]+128)/383;patch([0 1 1 0],[0 0 1 1],c1);patch([0 1 1 1-e 1-e 0+e],[0 0 1 1-e 0+e 0+e],c2);patch([0 0 1 1-e 0+e 0+e],[0 1 1 1-e 1-e 0+e],c3);plot([0 1 1 0 0],[0 0 1 1 0]);disp('Weights');
  "IW{1,2}(45,:)'" : Constant  Value=[0.06563629442723693807604234962127520702779293060302734375;0.37819706688799514804344426011084578931331634521484375;-0.3109773356045206771369748821598477661609649658203125;0.3830489996725623402795690708444453775882720947265625;0.25807245818522550617757360669202171266078948974609375;-0.0023620568424722009071015094150425284169614315032958984375;0.0164247632519410984019980759285317617468535900115966796875;-0.3175291683973353595860089626512490212917327880859375;-0.1424539759119330117886903508406248874962329864501953125;-0.355712659745710590986078614150756038725376129150390625]
      mask Display: e = 0.06;c1 = [120 150 230]/255;c2 = ([120 150 230]+0)/383;c3 = ([120 150 230]+128)/383;patch([0 1 1 0],[0 0 1 1],c1);patch([0 1 1 1-e 1-e 0+e],[0 0 1 1-e 0+e 0+e],c2);patch([0 0 1 1-e 0+e 0+e],[0 1 1 1-e 1-e 0+e],c3);plot([0 1 1 0 0],[0 0 1 1 0]);disp('Weights');
  "IW{1,2}(46,:)'" : Constant  Value=[-0.7599242403201496021125649349414743483066558837890625;0.311245626707613298744803387307911179959774017333984375;0.4513301182767204267065608291886746883392333984375;-0.349105266224237931194096518083824776113033294677734375;-0.326415196854076439247904772855690680444240570068359375;0.133872720375285247929042498071794398128986358642578125;0.1479321643633239313775362688829773105680942535400390625;0.0690960871733121706483871093951165676116943359375;0.00748656824979148337317891304110162309370934963226318359375;0.05862141364747007477031814914880669675767421722412109375]
      mask Display: e = 0.06;c1 = [120 150 230]/255;c2 = ([120 150 230]+0)/383;c3 = ([120 150 230]+128)/383;patch([0 1 1 0],[0 0 1 1],c1);patch([0 1 1 1-e 1-e 0+e],[0 0 1 1-e 0+e 0+e],c2);patch([0 0 1 1-e 0+e 0+e],[0 1 1 1-e 1-e 0+e],c3);plot([0 1 1 0 0],[0 0 1 1 0]);disp('Weights');
  "IW{1,2}(47,:)'" : Constant  Value=[0.641752566900068988076100140460766851902008056640625;0.46396433157034755456749053337262012064456939697265625;-0.166504348181084782520855469556408934295177459716796875;-0.067997156009429848833036658106721006333827972412109375;-0.34462816799041195992003849823959171772003173828125;-0.09343619402216431224506010266850353218615055084228515625;0.1527530649089583747457510298772831447422504425048828125;0.0204005276144635545876315774194154073484241962432861328125;-0.09926308259501992470319464700878597795963287353515625;-0.11300737519228508387580944827277562581002712249755859375]
      mask Display: e = 0.06;c1 = [120 150 230]/255;c2 = ([120 150 230]+0)/383;c3 = ([120 150 230]+128)/383;patch([0 1 1 0],[0 0 1 1],c1);patch([0 1 1 1-e 1-e 0+e],[0 0 1 1-e 0+e 0+e],c2);patch([0 0 1 1-e 0+e 0+e],[0 1 1 1-e 1-e 0+e],c3);plot([0 1 1 0 0],[0 0 1 1 0]);disp('Weights');
  "IW{1,2}(48,:)'" : Constant  Value=[0.6286915239198034299761275178752839565277099609375;-0.0923094741738320345714186032637371681630611419677734375;-0.525667897135358774818314486765302717685699462890625;-0.34634196476031398059802768329973332583904266357421875;0.2088975012705418798919509981715236790478229522705078125;0.3189078066195403238225480890832841396331787109375;0.3403261213552808417404094143421389162540435791015625;0.094058258439700559438989557747845537960529327392578125;0.25367785023551780998474214356974698603153228759765625;0.6423720397631289547035748910275287926197052001953125]
      mask Display: e = 0.06;c1 = [120 150 230]/255;c2 = ([120 150 230]+0)/383;c3 = ([120 150 230]+128)/383;patch([0 1 1 0],[0 0 1 1],c1);patch([0 1 1 1-e 1-e 0+e],[0 0 1 1-e 0+e 0+e],c2);patch([0 0 1 1-e 0+e 0+e],[0 1 1 1-e 1-e 0+e],c3);plot([0 1 1 0 0],[0 0 1 1 0]);disp('Weights');
  "IW{1,2}(49,:)'" : Constant  Value=[0.00783110948902149793526827892264918773435056209564208984375;0.074031369192252560740286071450100280344486236572265625;-0.06594149006553172431832621214198297820985317230224609375;-0.049279242551752831802414078765650629065930843353271484375;-0.026234103443511729014669953130578505806624889373779296875;-0.0134209267211293122035176139661416527815163135528564453125;-0.0281590194283356277937802047972581931389868259429931640625;0.027927253735328012862471069865932804532349109649658203125;0.0021400920173110689337381273844584939070045948028564453125;0.01877513474526958103805185373857966624200344085693359375]
      mask Display: e = 0.06;c1 = [120 150 230]/255;c2 = ([120 150 230]+0)/383;c3 = ([120 150 230]+128)/383;patch([0 1 1 0],[0 0 1 1],c1);patch([0 1 1 1-e 1-e 0+e],[0 0 1 1-e 0+e 0+e],c2);patch([0 0 1 1-e 0+e 0+e],[0 1 1 1-e 1-e 0+e],c3);plot([0 1 1 0 0],[0 0 1 1 0]);disp('Weights');
  "IW{1,2}(5,:)'" : Constant  Value=[-0.00801233294552941392729916714188220794312655925750732421875;-0.07520162066456871630126812533490010537207126617431640625;0.0668780520356412611082674857243546284735202789306640625;0.049972253706234648351625082796090282499790191650390625;0.026602236481148712476940687565729604102671146392822265625;0.0136099768024475036021225804461209918372333049774169921875;0.02856019843938605029531885293181403540074825286865234375;-0.0283886932248070926465555174900146084837615489959716796875;-0.0021945498145465127705355801168707330361939966678619384765625;-0.019081380097620094515864508366576046682894229888916015625]
      mask Display: e = 0.06;c1 = [120 150 230]/255;c2 = ([120 150 230]+0)/383;c3 = ([120 150 230]+128)/383;patch([0 1 1 0],[0 0 1 1],c1);patch([0 1 1 1-e 1-e 0+e],[0 0 1 1-e 0+e 0+e],c2);patch([0 0 1 1-e 0+e 0+e],[0 1 1 1-e 1-e 0+e],c3);plot([0 1 1 0 0],[0 0 1 1 0]);disp('Weights');
  "IW{1,2}(50,:)'" : Constant  Value=[0.04587112345533893298377137170973583124577999114990234375;0.102495986757728141380852093789144419133663177490234375;-0.1210533897694758553864602390603977255523204803466796875;0.041216737926025238947236317699207575060427188873291015625;-0.00420419844531171905954725076526301563717424869537353515625;0.11742829263354166713373416541799088008701801300048828125;0.06613098545981598019860570047967485152184963226318359375;-0.1053879141218486414910415760459727607667446136474609375;0.0142281809329760818016996637425108929164707660675048828125;0.09545103750455881386205447824977454729378223419189453125]
      mask Display: e = 0.06;c1 = [120 150 230]/255;c2 = ([120 150 230]+0)/383;c3 = ([120 150 230]+128)/383;patch([0 1 1 0],[0 0 1 1],c1);patch([0 1 1 1-e 1-e 0+e],[0 0 1 1-e 0+e 0+e],c2);patch([0 0 1 1-e 0+e 0+e],[0 1 1 1-e 1-e 0+e],c3);plot([0 1 1 0 0],[0 0 1 1 0]);disp('Weights');
  "IW{1,2}(51,:)'" : Constant  Value=[0.2387273994433078971866279971436597406864166259765625;-0.00415256252339484856206386353960624546743929386138916015625;-0.1823895595057546115125290953073999844491481781005859375;-0.2404200634657055191123475879066972993314266204833984375;-0.1758207127865518970555314126613666303455829620361328125;-0.317659663486635379658906686017871834337711334228515625;0.000400297449155439057956462622911431026295758783817291259765625;-0.1092129714237961568557011560187675058841705322265625;-0.315564834936291671585451013015699572861194610595703125;-0.37927367789468202641245397899183444678783416748046875]
      mask Display: e = 0.06;c1 = [120 150 230]/255;c2 = ([120 150 230]+0)/383;c3 = ([120 150 230]+128)/383;patch([0 1 1 0],[0 0 1 1],c1);patch([0 1 1 1-e 1-e 0+e],[0 0 1 1-e 0+e 0+e],c2);patch([0 0 1 1-e 0+e 0+e],[0 1 1 1-e 1-e 0+e],c3);plot([0 1 1 0 0],[0 0 1 1 0]);disp('Weights');
  "IW{1,2}(52,:)'" : Constant  Value=[-0.5456345059190306212570931165828369557857513427734375;0.336580832127757967331405097866081632673740386962890625;0.333552263557535144666843507366138510406017303466796875;-0.3965929917272177362974616698920726776123046875;-0.359121584020160644623587131718522869050502777099609375;0.3317527056262379314688359954743646085262298583984375;0.438933532281830796062394028922426514327526092529296875;0.0847029401898093947664847291889600455760955810546875;-0.3978526081459203833645688064279966056346893310546875;-0.432851432338583475001314582186751067638397216796875]
      mask Display: e = 0.06;c1 = [120 150 230]/255;c2 = ([120 150 230]+0)/383;c3 = ([120 150 230]+128)/383;patch([0 1 1 0],[0 0 1 1],c1);patch([0 1 1 1-e 1-e 0+e],[0 0 1 1-e 0+e 0+e],c2);patch([0 0 1 1-e 0+e 0+e],[0 1 1 1-e 1-e 0+e],c3);plot([0 1 1 0 0],[0 0 1 1 0]);disp('Weights');
  "IW{1,2}(53,:)'" : Constant  Value=[0.02134319543330766288935507191126816906034946441650390625;0.0126647979815222126720453132975308108143508434295654296875;0.434009204142607962761957196562434546649456024169921875;-0.454152935554614833879583102316246367990970611572265625;-0.11463023260690917426440904591800062917172908782958984375;-0.54220475055219352622515316397766582667827606201171875;0.09271785515872597860376203016130602918565273284912109375;0.04839962870916179882296859204870997928082942962646484375;0.304425936867545043895688650081865489482879638671875;0.3205679640209402325723431204096414148807525634765625]
      mask Display: e = 0.06;c1 = [120 150 230]/255;c2 = ([120 150 230]+0)/383;c3 = ([120 150 230]+128)/383;patch([0 1 1 0],[0 0 1 1],c1);patch([0 1 1 1-e 1-e 0+e],[0 0 1 1-e 0+e 0+e],c2);patch([0 0 1 1-e 0+e 0+e],[0 1 1 1-e 1-e 0+e],c3);plot([0 1 1 0 0],[0 0 1 1 0]);disp('Weights');
  "IW{1,2}(54,:)'" : Constant  Value=[0.2315364856389701408989623132583801634609699249267578125;0.0899495282188080835794607992283999919891357421875;0.139386741858552876127674835515790618956089019775390625;-0.029327407228733538835374616837725625373423099517822265625;0.10465403692043129257882583260652609169483184814453125;-0.1450488583513764029309101033504703082144260406494140625;0.1670683283051941636632165000264649279415607452392578125;-0.007904993108840692450645093458660994656383991241455078125;0.0176673944312657205113481495573068968951702117919921875;-0.08430813677339764333762417436446412466466426849365234375]
      mask Display: e = 0.06;c1 = [120 150 230]/255;c2 = ([120 150 230]+0)/383;c3 = ([120 150 230]+128)/383;patch([0 1 1 0],[0 0 1 1],c1);patch([0 1 1 1-e 1-e 0+e],[0 0 1 1-e 0+e 0+e],c2);patch([0 0 1 1-e 0+e 0+e],[0 1 1 1-e 1-e 0+e],c3);plot([0 1 1 0 0],[0 0 1 1 0]);disp('Weights');
  "IW{1,2}(55,:)'" : Constant  Value=[-0.01009305824310610839866786392349240486510097980499267578125;-0.08194646884067431635845224491276894696056842803955078125;0.07308142019900755459449470663457759656012058258056640625;0.054961818994648241332168225881105172447860240936279296875;0.0305027359921078260185378638880138169042766094207763671875;0.0164685100418424414103757413840867229737341403961181640625;0.032293363089086236927816031538895913399755954742431640625;-0.0298910622616588399214077043097859132103621959686279296875;-0.000749285680339964086336956849976331795915029942989349365234375;-0.0195446095230372880735547624908576835878193378448486328125]
      mask Display: e = 0.06;c1 = [120 150 230]/255;c2 = ([120 150 230]+0)/383;c3 = ([120 150 230]+128)/383;patch([0 1 1 0],[0 0 1 1],c1);patch([0 1 1 1-e 1-e 0+e],[0 0 1 1-e 0+e 0+e],c2);patch([0 0 1 1-e 0+e 0+e],[0 1 1 1-e 1-e 0+e],c3);plot([0 1 1 0 0],[0 0 1 1 0]);disp('Weights');
  "IW{1,2}(56,:)'" : Constant  Value=[-0.0079601368860716496811402720368278096430003643035888671875;-0.0748691664087833552709838613736792467534542083740234375;0.06660895165035206344494866925742826424539089202880859375;0.049772253192793165788021525486328755505383014678955078125;0.0264939457435163540355294031769517459906637668609619140625;0.0135524629523389138208155912934671505354344844818115234375;0.02844251497349893631483297440354363061487674713134765625;-0.028259660889887357193561712165319477207958698272705078125;-0.002182492354442170344464013709284699871204793453216552734375;-0.0189969581126583526853313088622599025256931781768798828125]
      mask Display: e = 0.06;c1 = [120 150 230]/255;c2 = ([120 150 230]+0)/383;c3 = ([120 150 230]+128)/383;patch([0 1 1 0],[0 0 1 1],c1);patch([0 1 1 1-e 1-e 0+e],[0 0 1 1-e 0+e 0+e],c2);patch([0 0 1 1-e 0+e 0+e],[0 1 1 1-e 1-e 0+e],c3);plot([0 1 1 0 0],[0 0 1 1 0]);disp('Weights');
  "IW{1,2}(57,:)'" : Constant  Value=[-0.9240574056008024061981132035725750029087066650390625;-0.235051001672422266164375059815938584506511688232421875;0.6786545452033403424962898498051799833774566650390625;-0.1451895390724890766431798283520038239657878875732421875;0.329777047621199581595163863312336616218090057373046875;-0.09084872424370293853002067407942377030849456787109375;-0.00373585280398288678560536624218002543784677982330322265625;-0.07414170693756548524699923063963069580495357513427734375;-0.3373521618354693440977598584140650928020477294921875;-0.281065689804717633304420587592176161706447601318359375]
      mask Display: e = 0.06;c1 = [120 150 230]/255;c2 = ([120 150 230]+0)/383;c3 = ([120 150 230]+128)/383;patch([0 1 1 0],[0 0 1 1],c1);patch([0 1 1 1-e 1-e 0+e],[0 0 1 1-e 0+e 0+e],c2);patch([0 0 1 1-e 0+e 0+e],[0 1 1 1-e 1-e 0+e],c3);plot([0 1 1 0 0],[0 0 1 1 0]);disp('Weights');
  "IW{1,2}(58,:)'" : Constant  Value=[0.0137833472798940710746240512207805295474827289581298828125;0.2606731672821080980639862900716252624988555908203125;0.21684913401635130814071317217894829809665679931640625;0.0570408891891254210548822811688296496868133544921875;0.1754733489816609759426313530639163218438625335693359375;-0.10645921084077192286798663189983926713466644287109375;0.005724025333909694805700762998412756132893264293670654296875;0.11037747686182523831899260358113679103553295135498046875;-0.046107003413617668463597709660461987368762493133544921875;0.28022159360404341743588929602992720901966094970703125]
      mask Display: e = 0.06;c1 = [120 150 230]/255;c2 = ([120 150 230]+0)/383;c3 = ([120 150 230]+128)/383;patch([0 1 1 0],[0 0 1 1],c1);patch([0 1 1 1-e 1-e 0+e],[0 0 1 1-e 0+e 0+e],c2);patch([0 0 1 1-e 0+e 0+e],[0 1 1 1-e 1-e 0+e],c3);plot([0 1 1 0 0],[0 0 1 1 0]);disp('Weights');
  "IW{1,2}(59,:)'" : Constant  Value=[0.1374566444496357620064230786738335154950618743896484375;-0.1157220185115146182663892204800504259765148162841796875;0.26372810911738231443024460531887598335742950439453125;-0.3368392831515214513871114831999875605106353759765625;0.13819687465548025073758253711275756359100341796875;-0.241125396208886566551399255331489257514476776123046875;-0.04557436446352140790860829611119697801768779754638671875;-0.00914631971451421686702953905978574766777455806732177734375;0.02513869109511490673725120359449647367000579833984375;0.07582269576512164210857491752904024906456470489501953125]
      mask Display: e = 0.06;c1 = [120 150 230]/255;c2 = ([120 150 230]+0)/383;c3 = ([120 150 230]+128)/383;patch([0 1 1 0],[0 0 1 1],c1);patch([0 1 1 1-e 1-e 0+e],[0 0 1 1-e 0+e 0+e],c2);patch([0 0 1 1-e 0+e 0+e],[0 1 1 1-e 1-e 0+e],c3);plot([0 1 1 0 0],[0 0 1 1 0]);disp('Weights');
  "IW{1,2}(6,:)'" : Constant  Value=[0.006450335888016626127716701688541434123180806636810302734375;0.0647505012906349486367929557673051021993160247802734375;-0.058817527542587122457717896395479328930377960205078125;-0.044087152705087902238023644940767553634941577911376953125;-0.0236762154347815341470795402756266412325203418731689453125;-0.01229887531518985936684895676762607763521373271942138671875;-0.025343735586211620092189633624002453871071338653564453125;0.0240716102107036040991250303022752632386982440948486328125;0.00137699656764471932944571275214684646925888955593109130859375;0.016098858234747492890193143466603942215442657470703125]
      mask Display: e = 0.06;c1 = [120 150 230]/255;c2 = ([120 150 230]+0)/383;c3 = ([120 150 230]+128)/383;patch([0 1 1 0],[0 0 1 1],c1);patch([0 1 1 1-e 1-e 0+e],[0 0 1 1-e 0+e 0+e],c2);patch([0 0 1 1-e 0+e 0+e],[0 1 1 1-e 1-e 0+e],c3);plot([0 1 1 0 0],[0 0 1 1 0]);disp('Weights');
  "IW{1,2}(60,:)'" : Constant  Value=[0.0055471269580359694462146080695674754679203033447265625;0.05854176590173883198975346431325306184589862823486328125;-0.05406284868909605467734991179895587265491485595703125;-0.0406195954027717409662301406569895334541797637939453125;-0.0219983393492985922212934468689127243123948574066162109375;-0.01159058496105492240546563920133849023841321468353271484375;-0.0234885040822550884842545571018490591086447238922119140625;0.0214779415191480756164299492638747324235737323760986328125;0.00083659667252587721630874284528545103967189788818359375;0.01429071273310309093951264713950877194292843341827392578125]
      mask Display: e = 0.06;c1 = [120 150 230]/255;c2 = ([120 150 230]+0)/383;c3 = ([120 150 230]+128)/383;patch([0 1 1 0],[0 0 1 1],c1);patch([0 1 1 1-e 1-e 0+e],[0 0 1 1-e 0+e 0+e],c2);patch([0 0 1 1-e 0+e 0+e],[0 1 1 1-e 1-e 0+e],c3);plot([0 1 1 0 0],[0 0 1 1 0]);disp('Weights');
  "IW{1,2}(61,:)'" : Constant  Value=[-0.53606944945962109461135014498722739517688751220703125;-0.0830241725110067718684803139694849960505962371826171875;-0.75443150032839145779917089384980499744415283203125;0.340095781232454374976015287757036276161670684814453125;0.30872404606029579809955976088531315326690673828125;0.285744889265579893322666293897782452404499053955078125;0.360099206842040608922417277426575310528278350830078125;-0.2026811064786902816248215231098583899438381195068359375;0.0750453315907615159385812830805662088096141815185546875;0.151791039693124851783778694880311377346515655517578125]
      mask Display: e = 0.06;c1 = [120 150 230]/255;c2 = ([120 150 230]+0)/383;c3 = ([120 150 230]+128)/383;patch([0 1 1 0],[0 0 1 1],c1);patch([0 1 1 1-e 1-e 0+e],[0 0 1 1-e 0+e 0+e],c2);patch([0 0 1 1-e 0+e 0+e],[0 1 1 1-e 1-e 0+e],c3);plot([0 1 1 0 0],[0 0 1 1 0]);disp('Weights');
  "IW{1,2}(62,:)'" : Constant  Value=[-0.00619601002820189920849980325101569178514182567596435546875;-0.0630114177595981483914755472142132930457592010498046875;0.0574898359684793691659621117651113308966159820556640625;0.043120190958495265010075314648929634131491184234619140625;0.0232085676481234744195081276529890601523220539093017578125;0.01210214818900105272769796016518739634193480014801025390625;0.024827145332792212306660672993530170060694217681884765625;-0.0233433762894651418429159406286999001167714595794677734375;-0.00122342594022647349095989088851865744800306856632232666015625;-0.01559044695096782097432086544586127274669706821441650390625]
      mask Display: e = 0.06;c1 = [120 150 230]/255;c2 = ([120 150 230]+0)/383;c3 = ([120 150 230]+128)/383;patch([0 1 1 0],[0 0 1 1],c1);patch([0 1 1 1-e 1-e 0+e],[0 0 1 1-e 0+e 0+e],c2);patch([0 0 1 1-e 0+e 0+e],[0 1 1 1-e 1-e 0+e],c3);plot([0 1 1 0 0],[0 0 1 1 0]);disp('Weights');
  "IW{1,2}(63,:)'" : Constant  Value=[-0.10899598156518598701669731099173077382147312164306640625;-0.38338791758090084993426671644556336104869842529296875;0.0946649833586936384488552675975370220839977264404296875;0.09731050329213837557507105202603270299732685089111328125;-0.054359892437083716376644559886699425987899303436279296875;-0.35367633474813320315632836354780010879039764404296875;-0.31759021228900718991638996158144436776638031005859375;-0.359423220623583394850442118695355020463466644287109375;0.039583397966895271513632081905598170123994350433349609375;-0.03578591740633675633009858074728981591761112213134765625]
      mask Display: e = 0.06;c1 = [120 150 230]/255;c2 = ([120 150 230]+0)/383;c3 = ([120 150 230]+128)/383;patch([0 1 1 0],[0 0 1 1],c1);patch([0 1 1 1-e 1-e 0+e],[0 0 1 1-e 0+e 0+e],c2);patch([0 0 1 1-e 0+e 0+e],[0 1 1 1-e 1-e 0+e],c3);plot([0 1 1 0 0],[0 0 1 1 0]);disp('Weights');
  "IW{1,2}(64,:)'" : Constant  Value=[0.03538323284052395656384959465867723338305950164794921875;-0.0234334058790095674240649969988226075656712055206298828125;-0.42643364114070114734289518310106359422206878662109375;-0.1154642896338170798831157526365132071077823638916015625;0.0734347540454273473020663232091465033590793609619140625;0.1432105764030799921471270863548852503299713134765625;0.2373997394507786073969413109807646833360195159912109375;-0.1340305425873167255446105627925135195255279541015625;0.14757511966163694427933705810573883354663848876953125;0.166998434214602031744334453833289444446563720703125]
      mask Display: e = 0.06;c1 = [120 150 230]/255;c2 = ([120 150 230]+0)/383;c3 = ([120 150 230]+128)/383;patch([0 1 1 0],[0 0 1 1],c1);patch([0 1 1 1-e 1-e 0+e],[0 0 1 1-e 0+e 0+e],c2);patch([0 0 1 1-e 0+e 0+e],[0 1 1 1-e 1-e 0+e],c3);plot([0 1 1 0 0],[0 0 1 1 0]);disp('Weights');
  "IW{1,2}(65,:)'" : Constant  Value=[0.10841242199356089515038803483548690564930438995361328125;0.0675547742727371780535605694240075536072254180908203125;0.137038573566636900924464725903817452490329742431640625;0.36468071405031532439267039080732502043247222900390625;0.366486629144569475702297722818912006914615631103515625;0.337861284676247375369229075658950023353099822998046875;-0.1189152256869487056523126966567360796034336090087890625;-0.137988181002448861978137983896885998547077178955078125;-0.12120846820254037312647454882608144544064998626708984375;-0.366735535715038973858526105686905793845653533935546875]
      mask Display: e = 0.06;c1 = [120 150 230]/255;c2 = ([120 150 230]+0)/383;c3 = ([120 150 230]+128)/383;patch([0 1 1 0],[0 0 1 1],c1);patch([0 1 1 1-e 1-e 0+e],[0 0 1 1-e 0+e 0+e],c2);patch([0 0 1 1-e 0+e 0+e],[0 1 1 1-e 1-e 0+e],c3);plot([0 1 1 0 0],[0 0 1 1 0]);disp('Weights');
  "IW{1,2}(66,:)'" : Constant  Value=[-0.348734486931703113743452604467165656387805938720703125;0.268744041330844563031376992512377910315990447998046875;0.1742988603789233092999921836963039822876453399658203125;-0.2306781715802361520939456340784090571105480194091796875;-0.2006065768255071990466831266530789434909820556640625;0.11314863663363418366802903847201378084719181060791015625;-0.257625635827576082714784888594294898211956024169921875;-0.237921603946771309523455784074030816555023193359375;-0.063236469011119178507129845456802286207675933837890625;-0.11474434283012026336567856787951313890516757965087890625]
      mask Display: e = 0.06;c1 = [120 150 230]/255;c2 = ([120 150 230]+0)/383;c3 = ([120 150 230]+128)/383;patch([0 1 1 0],[0 0 1 1],c1);patch([0 1 1 1-e 1-e 0+e],[0 0 1 1-e 0+e 0+e],c2);patch([0 0 1 1-e 0+e 0+e],[0 1 1 1-e 1-e 0+e],c3);plot([0 1 1 0 0],[0 0 1 1 0]);disp('Weights');
  "IW{1,2}(67,:)'" : Constant  Value=[-0.1413634945235867912405325341751449741423130035400390625;-0.17718575184882301432054418910411186516284942626953125;0.1392756329402569936970479602678096853196620941162109375;-0.005290470883346384996237521392004055087454617023468017578125;0.40228142354877782782551776108448393642902374267578125;0.354869022084309426734449743889854289591312408447265625;-0.0688696189066963782021701945268432609736919403076171875;0.022461421504704405516239518192378454841673374176025390625;-0.11409576252366725179765438724643900059163570404052734375;0.184000856085178854382178315063356421887874603271484375]
      mask Display: e = 0.06;c1 = [120 150 230]/255;c2 = ([120 150 230]+0)/383;c3 = ([120 150 230]+128)/383;patch([0 1 1 0],[0 0 1 1],c1);patch([0 1 1 1-e 1-e 0+e],[0 0 1 1-e 0+e 0+e],c2);patch([0 0 1 1-e 0+e 0+e],[0 1 1 1-e 1-e 0+e],c3);plot([0 1 1 0 0],[0 0 1 1 0]);disp('Weights');
  "IW{1,2}(68,:)'" : Constant  Value=[0.0700257505156910708965511958012939430773258209228515625;-0.293881051126017478480889622005634009838104248046875;-0.2131614825356262787892092092079110443592071533203125;0.5642235713089573945211441241553984582424163818359375;0.1630483113949482143478775242328993044793605804443359375;0.6689435152123888173036903026513755321502685546875;-0.127419347508939628799140564296976663172245025634765625;0.09368561333392581846890578844977426342666149139404296875;0.039210251806375939764848226332105696201324462890625;0.07418570426289795849417174622431048192083835601806640625]
      mask Display: e = 0.06;c1 = [120 150 230]/255;c2 = ([120 150 230]+0)/383;c3 = ([120 150 230]+128)/383;patch([0 1 1 0],[0 0 1 1],c1);patch([0 1 1 1-e 1-e 0+e],[0 0 1 1-e 0+e 0+e],c2);patch([0 0 1 1-e 0+e 0+e],[0 1 1 1-e 1-e 0+e],c3);plot([0 1 1 0 0],[0 0 1 1 0]);disp('Weights');
  "IW{1,2}(69,:)'" : Constant  Value=[-0.17225478928316173554691204117261804640293121337890625;0.04136361889152286031023919576909975148737430572509765625;-0.06792813701780235635663274251783150248229503631591796875;0.6373322164630554897968295335886068642139434814453125;-0.217858633751632335684433883216115646064281463623046875;0.2184348251170423471645420931963599286973476409912109375;0.23289858629858162242243224682169966399669647216796875;0.37898954404875995205514982444583438336849212646484375;0.1490379247013667585175511476336396299302577972412109375;-0.293229068949460380810734250189852900803089141845703125]
      mask Display: e = 0.06;c1 = [120 150 230]/255;c2 = ([120 150 230]+0)/383;c3 = ([120 150 230]+128)/383;patch([0 1 1 0],[0 0 1 1],c1);patch([0 1 1 1-e 1-e 0+e],[0 0 1 1-e 0+e 0+e],c2);patch([0 0 1 1-e 0+e 0+e],[0 1 1 1-e 1-e 0+e],c3);plot([0 1 1 0 0],[0 0 1 1 0]);disp('Weights');
  "IW{1,2}(7,:)'" : Constant  Value=[-0.00779042800484481927358881847567317890934646129608154296875;-0.073764247797119264493659329673391766846179962158203125;0.06573108488620944822589109435284626670181751251220703125;0.049124517432346616330196553690257132984697818756103515625;0.026154124205801564106987910918178386054933071136474609375;0.01338193915615334093904831291865775710903108119964599609375;0.028071529149404424174907290989722241647541522979736328125;-0.0278196942790493555175412865310136112384498119354248046875;-0.002123941912192028359795958891709233284927904605865478515625;-0.0187024151279206220233053414858659380115568637847900390625]
      mask Display: e = 0.06;c1 = [120 150 230]/255;c2 = ([120 150 230]+0)/383;c3 = ([120 150 230]+128)/383;patch([0 1 1 0],[0 0 1 1],c1);patch([0 1 1 1-e 1-e 0+e],[0 0 1 1-e 0+e 0+e],c2);patch([0 0 1 1-e 0+e 0+e],[0 1 1 1-e 1-e 0+e],c3);plot([0 1 1 0 0],[0 0 1 1 0]);disp('Weights');
  "IW{1,2}(70,:)'" : Constant  Value=[0.00661505773533277267872687588123881141655147075653076171875;0.06587283751865082026544229165665456093847751617431640625;-0.059673448014316975152038224905481911264359951019287109375;-0.04471010675747062734775028047806699760258197784423828125;-0.023977774381534151804107324323922512121498584747314453125;-0.0124258578937376830408911843051100731827318668365478515625;-0.025676619354611192325155144544623908586800098419189453125;0.02454186821815675101365883392645628191530704498291015625;0.0014763640377913737379567127305790563696064054965972900390625;0.0164273241383162856010802244099977542646229267120361328125]
      mask Display: e = 0.06;c1 = [120 150 230]/255;c2 = ([120 150 230]+0)/383;c3 = ([120 150 230]+128)/383;patch([0 1 1 0],[0 0 1 1],c1);patch([0 1 1 1-e 1-e 0+e],[0 0 1 1-e 0+e 0+e],c2);patch([0 0 1 1-e 0+e 0+e],[0 1 1 1-e 1-e 0+e],c3);plot([0 1 1 0 0],[0 0 1 1 0]);disp('Weights');
  "IW{1,2}(71,:)'" : Constant  Value=[0.00856734842360248709247638743136121775023639202117919921875;0.0805211552355509507794550927428645081818103790283203125;-0.0707358759247143920045886034131399355828762054443359375;-0.052802839899786492561251094457475119270384311676025390625;-0.027846523517490680277308712220474262721836566925048828125;-0.01398500447484574658874034724931334494613111019134521484375;-0.0298661384514750764818113992760117980651557445526123046875;0.0308240321198023324578141313168089254759252071380615234375;0.0029266314388043369008884919679758240818046033382415771484375;0.0207754090007528924299862183033837936818599700927734375]
      mask Display: e = 0.06;c1 = [120 150 230]/255;c2 = ([120 150 230]+0)/383;c3 = ([120 150 230]+128)/383;patch([0 1 1 0],[0 0 1 1],c1);patch([0 1 1 1-e 1-e 0+e],[0 0 1 1-e 0+e 0+e],c2);patch([0 0 1 1-e 0+e 0+e],[0 1 1 1-e 1-e 0+e],c3);plot([0 1 1 0 0],[0 0 1 1 0]);disp('Weights');
  "IW{1,2}(72,:)'" : Constant  Value=[-0.10949718999100023497650369108669110573828220367431640625;-0.2941903442223254838694401769316755235195159912109375;-0.207423660958987898794703141902573406696319580078125;-0.1801758309294279047918507785652764141559600830078125;-0.299656438307677797094896732232882641255855560302734375;-0.1024800888478863691855025308541371487081050872802734375;0.2212918490883914734990156603089417330920696258544921875;0.0981645332169653606069203988226945511996746063232421875;0.092067304055237830784363950442639179527759552001953125;-0.1471544847929217303406090877615497447550296783447265625]
      mask Display: e = 0.06;c1 = [120 150 230]/255;c2 = ([120 150 230]+0)/383;c3 = ([120 150 230]+128)/383;patch([0 1 1 0],[0 0 1 1],c1);patch([0 1 1 1-e 1-e 0+e],[0 0 1 1-e 0+e 0+e],c2);patch([0 0 1 1-e 0+e 0+e],[0 1 1 1-e 1-e 0+e],c3);plot([0 1 1 0 0],[0 0 1 1 0]);disp('Weights');
  "IW{1,2}(73,:)'" : Constant  Value=[0.00619377737609348721914415136780007742345333099365234375;0.0629961186040937926033933536018594168126583099365234375;-0.057478145294033979040282389405547291971743106842041015625;-0.043111672615652428530719220134415081702172756195068359375;-0.02320444882004812914289004766033031046390533447265625;-0.012100414925658477260927980978522100485861301422119140625;-0.0248225935625863251832168288046887028031051158905029296875;0.0233369738982593007137200658007714082486927509307861328125;0.00122207966707225880627352143648067794856615364551544189453125;0.0155859790920187570029131762794349924661219120025634765625]
      mask Display: e = 0.06;c1 = [120 150 230]/255;c2 = ([120 150 230]+0)/383;c3 = ([120 150 230]+128)/383;patch([0 1 1 0],[0 0 1 1],c1);patch([0 1 1 1-e 1-e 0+e],[0 0 1 1-e 0+e 0+e],c2);patch([0 0 1 1-e 0+e 0+e],[0 1 1 1-e 1-e 0+e],c3);plot([0 1 1 0 0],[0 0 1 1 0]);disp('Weights');
  "IW{1,2}(74,:)'" : Constant  Value=[0.00796283251811428192945552240189499570988118648529052734375;0.074886451927383468341048455840791575610637664794921875;-0.0666228745686030798811572140039061196148395538330078125;-0.049782581071489868940194156721190665848553180694580078125;-0.0264994907925405580317868015072235721163451671600341796875;-0.01355536574916115476197031597394015989266335964202880859375;-0.028448548854529513707500854025056469254195690155029296875;0.0282664173157827249005524805625100270844995975494384765625;0.0021831979728401339733989683367099132738076150417327880859375;0.0190014068617429289498321764995125704444944858551025390625]
      mask Display: e = 0.06;c1 = [120 150 230]/255;c2 = ([120 150 230]+0)/383;c3 = ([120 150 230]+128)/383;patch([0 1 1 0],[0 0 1 1],c1);patch([0 1 1 1-e 1-e 0+e],[0 0 1 1-e 0+e 0+e],c2);patch([0 0 1 1-e 0+e 0+e],[0 1 1 1-e 1-e 0+e],c3);plot([0 1 1 0 0],[0 0 1 1 0]);disp('Weights');
  "IW{1,2}(75,:)'" : Constant  Value=[-0.307734176432365946762814701287425123155117034912109375;-0.1286169436302920521253412289297557435929775238037109375;0.0128343455476772443091260100800354848615825176239013671875;0.238880027745760725732537821386358700692653656005859375;-0.324733369235029101229628167857299558818340301513671875;-0.043018970852601430554518202598046627826988697052001953125;-0.3787219238720374026030413006083108484745025634765625;-0.194347652908113233127807006894727237522602081298828125;-0.20620012345346150350877678647520951926708221435546875;0.26268888807607027047197334468364715576171875]
      mask Display: e = 0.06;c1 = [120 150 230]/255;c2 = ([120 150 230]+0)/383;c3 = ([120 150 230]+128)/383;patch([0 1 1 0],[0 0 1 1],c1);patch([0 1 1 1-e 1-e 0+e],[0 0 1 1-e 0+e 0+e],c2);patch([0 0 1 1-e 0+e 0+e],[0 1 1 1-e 1-e 0+e],c3);plot([0 1 1 0 0],[0 0 1 1 0]);disp('Weights');
  "IW{1,2}(76,:)'" : Constant  Value=[0.13849101833063082178654212839319370687007904052734375;-0.05314914385130535545709307143624755553901195526123046875;0.497122642672203018943122287964797578752040863037109375;0.4110924394139150450655506574548780918121337890625;0.2290434115684903126908267267936025746166706085205078125;0.06872317245472493729696594755296246148645877838134765625;0.1508650196702952805960507021154626272618770599365234375;-0.03926928713022224959328099203048623166978359222412109375;0.04652758211313645642093206333811394870281219482421875;-0.032724594777101066733759893168098642490804195404052734375]
      mask Display: e = 0.06;c1 = [120 150 230]/255;c2 = ([120 150 230]+0)/383;c3 = ([120 150 230]+128)/383;patch([0 1 1 0],[0 0 1 1],c1);patch([0 1 1 1-e 1-e 0+e],[0 0 1 1-e 0+e 0+e],c2);patch([0 0 1 1-e 0+e 0+e],[0 1 1 1-e 1-e 0+e],c3);plot([0 1 1 0 0],[0 0 1 1 0]);disp('Weights');
  "IW{1,2}(77,:)'" : Constant  Value=[0.005574113616244929549081721376069253892637789249420166015625;0.058728606689789540629131892046643770299851894378662109375;-0.05420665289295367728072960744611918926239013671875;-0.040724680326161950827401625474522006697952747344970703125;-0.0220492819712536126941504477372291148640215396881103515625;-0.01161224825351592215838536503724753856658935546875;-0.0235448929700899332873031966073540388606488704681396484375;0.0215556748283516376452073615155313746072351932525634765625;0.000852442945711465106979620731664226696011610329151153564453125;0.0143447791513248400219193712246124050579965114593505859375]
      mask Display: e = 0.06;c1 = [120 150 230]/255;c2 = ([120 150 230]+0)/383;c3 = ([120 150 230]+128)/383;patch([0 1 1 0],[0 0 1 1],c1);patch([0 1 1 1-e 1-e 0+e],[0 0 1 1-e 0+e 0+e],c2);patch([0 0 1 1-e 0+e 0+e],[0 1 1 1-e 1-e 0+e],c3);plot([0 1 1 0 0],[0 0 1 1 0]);disp('Weights');
  "IW{1,2}(78,:)'" : Constant  Value=[0.00778986147982392573840826344166998751461505889892578125;0.07376052036204695794285868259976268745958805084228515625;-0.06572815645568723386116261053757625631988048553466796875;-0.049122366099054660948386441532420576550066471099853515625;-0.0261530169622286035036040630075149238109588623046875;-0.01338140417814025033560465516302429023198783397674560546875;-0.028070317282863473107301643949540448375046253204345703125;0.027818188533738776035963979893494979478418827056884765625;0.002123708470767689780733800120060550398193299770355224609375;0.0187013942688763375177263270643379655666649341583251953125]
      mask Display: e = 0.06;c1 = [120 150 230]/255;c2 = ([120 150 230]+0)/383;c3 = ([120 150 230]+128)/383;patch([0 1 1 0],[0 0 1 1],c1);patch([0 1 1 1-e 1-e 0+e],[0 0 1 1-e 0+e 0+e],c2);patch([0 0 1 1-e 0+e 0+e],[0 1 1 1-e 1-e 0+e],c3);plot([0 1 1 0 0],[0 0 1 1 0]);disp('Weights');
  "IW{1,2}(79,:)'" : Constant  Value=[-0.007669272951113287502267201745098645915277302265167236328125;-0.07296390571697948523866017467298661358654499053955078125;0.0651055183839352180630299926633597351610660552978515625;0.048665859773598545146011673523389617912471294403076171875;0.0259201444044292912682880825059328344650566577911376953125;0.0132709621382449578785855948126481962390244007110595703125;0.0278151490549122422379912933365631033666431903839111328125;-0.0274943561290978688571584598321351222693920135498046875;-0.0020703849502057354754758211612397644785232841968536376953125;-0.0184806142730388443806699427796047530137002468109130859375]
      mask Display: e = 0.06;c1 = [120 150 230]/255;c2 = ([120 150 230]+0)/383;c3 = ([120 150 230]+128)/383;patch([0 1 1 0],[0 0 1 1],c1);patch([0 1 1 1-e 1-e 0+e],[0 0 1 1-e 0+e 0+e],c2);patch([0 0 1 1-e 0+e 0+e],[0 1 1 1-e 1-e 0+e],c3);plot([0 1 1 0 0],[0 0 1 1 0]);disp('Weights');
  "IW{1,2}(8,:)'" : Constant  Value=[-0.008313732556325191536128471625488600693643093109130859375;-0.0769263054143709823495811406246502883732318878173828125;0.068345574737835701473187555166077800095081329345703125;0.051085047184044031498562077331371256150305271148681640625;0.02726221838423707743981339035599376074969768524169921875;0.01400841354140890289425858128424806636758148670196533203125;0.029264535076659027590384454242666834034025669097900390625;-0.0290019931491190853523054471452269353903830051422119140625;-0.0021656411364033623968838870865738499560393393039703369140625;-0.01945110719536731480605595834276755340397357940673828125]
      mask Display: e = 0.06;c1 = [120 150 230]/255;c2 = ([120 150 230]+0)/383;c3 = ([120 150 230]+128)/383;patch([0 1 1 0],[0 0 1 1],c1);patch([0 1 1 1-e 1-e 0+e],[0 0 1 1-e 0+e 0+e],c2);patch([0 0 1 1-e 0+e 0+e],[0 1 1 1-e 1-e 0+e],c3);plot([0 1 1 0 0],[0 0 1 1 0]);disp('Weights');
  "IW{1,2}(80,:)'" : Constant  Value=[0.00866304211342162899800456443699658848345279693603515625;0.07959986419815578972958292069961316883563995361328125;-0.0705283139969269112778960106879821978509426116943359375;-0.052745798028333977514048314105821191333234310150146484375;-0.0281717302729052911092200162102017202414572238922119140625;-0.01449933846294436390333970621213666163384914398193359375;-0.0302255867905414886409598551608723937533795833587646484375;0.0300666835483465212652820497396533028222620487213134765625;0.0022709535248286688395580323884814788470976054668426513671875;0.020111919562960524354711111527649336494505405426025390625]
      mask Display: e = 0.06;c1 = [120 150 230]/255;c2 = ([120 150 230]+0)/383;c3 = ([120 150 230]+128)/383;patch([0 1 1 0],[0 0 1 1],c1);patch([0 1 1 1-e 1-e 0+e],[0 0 1 1-e 0+e 0+e],c2);patch([0 0 1 1-e 0+e 0+e],[0 1 1 1-e 1-e 0+e],c3);plot([0 1 1 0 0],[0 0 1 1 0]);disp('Weights');
  "IW{1,2}(81,:)'" : Constant  Value=[-0.0078378044837576731074246794150894857011735439300537109375;-0.07407522641225740278603240085431025363504886627197265625;0.06597612814385989121745978991384617984294891357421875;0.04930474080098067035660136525621055625379085540771484375;0.02624734420335668449997257312134024687111377716064453125;0.0134274406363567265498826230896156630478799343109130859375;0.028173494976577888315727449253245140425860881805419921875;-0.0279448536556729208724103585836928687058389186859130859375;-0.00214264347637391390499761456567284767515957355499267578125;-0.0187869982061720126875759007134547573514282703399658203125]
      mask Display: e = 0.06;c1 = [120 150 230]/255;c2 = ([120 150 230]+0)/383;c3 = ([120 150 230]+128)/383;patch([0 1 1 0],[0 0 1 1],c1);patch([0 1 1 1-e 1-e 0+e],[0 0 1 1-e 0+e 0+e],c2);patch([0 0 1 1-e 0+e 0+e],[0 1 1 1-e 1-e 0+e],c3);plot([0 1 1 0 0],[0 0 1 1 0]);disp('Weights');
  "IW{1,2}(82,:)'" : Constant  Value=[-0.00849789047607767307479509355516711366362869739532470703125;-0.07770128606153527128785896138651878573000431060791015625;0.0690635081289484309419179908218211494386196136474609375;0.051649989837669836589828520345690776593983173370361328125;0.0276594445658981842595114386540444684214890003204345703125;0.01428874829386965646105256411146910977549850940704345703125;0.0296690258961389875802527882342474185861647129058837890625;-0.0292170343451981680271689612027330440469086170196533203125;-0.002056323516251346884831097128198962309397757053375244140625;-0.0195464462250868990789154366893853875808417797088623046875]
      mask Display: e = 0.06;c1 = [120 150 230]/255;c2 = ([120 150 230]+0)/383;c3 = ([120 150 230]+128)/383;patch([0 1 1 0],[0 0 1 1],c1);patch([0 1 1 1-e 1-e 0+e],[0 0 1 1-e 0+e 0+e],c2);patch([0 0 1 1-e 0+e 0+e],[0 1 1 1-e 1-e 0+e],c3);plot([0 1 1 0 0],[0 0 1 1 0]);disp('Weights');
  "IW{1,2}(83,:)'" : Constant  Value=[-0.00829318650636188918479074771994419279508292675018310546875;-0.07682521247041386447396149605992832221090793609619140625;0.0682549143437376215626244402301381342113018035888671875;0.051014815615542281890260056798069854266941547393798828125;0.027216405744303472091782936104209511540830135345458984375;0.01397784265785556763461716656138378311879932880401611328125;0.029216738173555807656089911006347392685711383819580078125;-0.0289702103828696488907468165052705444395542144775390625;-0.002174048169437101975243198381804177188314497470855712890625;-0.019434400615108649024165288210497237741947174072265625]
      mask Display: e = 0.06;c1 = [120 150 230]/255;c2 = ([120 150 230]+0)/383;c3 = ([120 150 230]+128)/383;patch([0 1 1 0],[0 0 1 1],c1);patch([0 1 1 1-e 1-e 0+e],[0 0 1 1-e 0+e 0+e],c2);patch([0 0 1 1-e 0+e 0+e],[0 1 1 1-e 1-e 0+e],c3);plot([0 1 1 0 0],[0 0 1 1 0]);disp('Weights');
  "IW{1,2}(84,:)'" : Constant  Value=[-0.49368229820591980061550430036731995642185211181640625;-0.45898684946655665672921031728037633001804351806640625;-0.0762255724241505394633833248008158989250659942626953125;-0.05395222340349768719303114039576030336320400238037109375;0.36559230440862855449069002133910544216632843017578125;0.05339374248459594074489587001153267920017242431640625;0.32768687612741675962979570613242685794830322265625;0.2243970173181835392473004731073160655796527862548828125;0.06617409755495211320930337706158752553164958953857421875;0.07606370405053641814419052025186829268932342529296875]
      mask Display: e = 0.06;c1 = [120 150 230]/255;c2 = ([120 150 230]+0)/383;c3 = ([120 150 230]+128)/383;patch([0 1 1 0],[0 0 1 1],c1);patch([0 1 1 1-e 1-e 0+e],[0 0 1 1-e 0+e 0+e],c2);patch([0 0 1 1-e 0+e 0+e],[0 1 1 1-e 1-e 0+e],c3);plot([0 1 1 0 0],[0 0 1 1 0]);disp('Weights');
  "IW{1,2}(85,:)'" : Constant  Value=[0.14914222283411315839174449138226918876171112060546875;-0.1939990862344092847902032872298150323331356048583984375;-0.12303110029121804014362595580678316764533519744873046875;0.01249102159560766533985542992013506591320037841796875;-0.1500344301176514127948991017547086812555789947509765625;-0.38761520255203507634433890416403301060199737548828125;-0.357134400291312215092176529651624150574207305908203125;-0.287148460068477884288284940339508466422557830810546875;0.0239381050403746804822180394012320903129875659942626953125;0.08111377992136166448222667213485692627727985382080078125]
      mask Display: e = 0.06;c1 = [120 150 230]/255;c2 = ([120 150 230]+0)/383;c3 = ([120 150 230]+128)/383;patch([0 1 1 0],[0 0 1 1],c1);patch([0 1 1 1-e 1-e 0+e],[0 0 1 1-e 0+e 0+e],c2);patch([0 0 1 1-e 0+e 0+e],[0 1 1 1-e 1-e 0+e],c3);plot([0 1 1 0 0],[0 0 1 1 0]);disp('Weights');
  "IW{1,2}(86,:)'" : Constant  Value=[-0.317465906880486203878177775550284422934055328369140625;0.006720809144096405278456796139607831719331443309783935546875;0.487793828059973788580094833378097973763942718505859375;-0.475027697625448663831804196888697333633899688720703125;0.08340188206273317639283249036452616564929485321044921875;0.254943238462851329284575285782921127974987030029296875;0.2338154291758578751103669901567627675831317901611328125;0.192261632399450543839947158630820922553539276123046875;0.061394976995939383457301374846792896278202533721923828125;0.0181331202606591183890127894073884817771613597869873046875]
      mask Display: e = 0.06;c1 = [120 150 230]/255;c2 = ([120 150 230]+0)/383;c3 = ([120 150 230]+128)/383;patch([0 1 1 0],[0 0 1 1],c1);patch([0 1 1 1-e 1-e 0+e],[0 0 1 1-e 0+e 0+e],c2);patch([0 0 1 1-e 0+e 0+e],[0 1 1 1-e 1-e 0+e],c3);plot([0 1 1 0 0],[0 0 1 1 0]);disp('Weights');
  "IW{1,2}(87,:)'" : Constant  Value=[-0.007853202365350246683117774182392167858779430389404296875;-0.07417597145132191760463769014677382074296474456787109375;0.0660558008244731820202133576458436436951160430908203125;0.049363420728680863780457599432338611222803592681884765625;0.02627788437280996480804873272063559852540493011474609375;0.0134425321997429236819954212478478439152240753173828125;0.0282068731033136392560844996069135959260165691375732421875;-0.02798521467414981367394233302547945640981197357177734375;-0.0021483904126659921114683715615001347032375633716583251953125;-0.01881416336463574701109990883196587674319744110107421875]
      mask Display: e = 0.06;c1 = [120 150 230]/255;c2 = ([120 150 230]+0)/383;c3 = ([120 150 230]+128)/383;patch([0 1 1 0],[0 0 1 1],c1);patch([0 1 1 1-e 1-e 0+e],[0 0 1 1-e 0+e 0+e],c2);patch([0 0 1 1-e 0+e 0+e],[0 1 1 1-e 1-e 0+e],c3);plot([0 1 1 0 0],[0 0 1 1 0]);disp('Weights');
  "IW{1,2}(88,:)'" : Constant  Value=[-0.007410892846253254624688810991983700660057365894317626953125;-0.0712430734091211437242208148745703510940074920654296875;0.0637760235358211247103099594824016094207763671875;0.04769528932651041774892775038097170181572437286376953125;0.0254350381486666658747974878451714175753295421600341796875;0.0130510524776014692760472968302565277554094791412353515625;0.027282286956901914687367849410293274559080600738525390625;-0.0267851563010616834648036643784507759846746921539306640625;-0.00193881307528575934882864029162874430767260491847991943359375;-0.0179913418424687866770117494752412312664091587066650390625]
      mask Display: e = 0.06;c1 = [120 150 230]/255;c2 = ([120 150 230]+0)/383;c3 = ([120 150 230]+128)/383;patch([0 1 1 0],[0 0 1 1],c1);patch([0 1 1 1-e 1-e 0+e],[0 0 1 1-e 0+e 0+e],c2);patch([0 0 1 1-e 0+e 0+e],[0 1 1 1-e 1-e 0+e],c3);plot([0 1 1 0 0],[0 0 1 1 0]);disp('Weights');
  "IW{1,2}(89,:)'" : Constant  Value=[-0.289837574843206879915413765047560445964336395263671875;-0.2238789851364168248526453908198163844645023345947265625;0.323471286455276840765549195566563867032527923583984375;-0.314633169648115218475226129157817922532558441162109375;-0.173460971696423105203876957602915354073047637939453125;-0.61336893868021402642654038572800345718860626220703125;-0.139813684582678454670912060464615933597087860107421875;0.0185728424138764565409775997295582783408463001251220703125;-0.25851629774593976041074938621022738516330718994140625;-0.113142465402051417555640000500716269016265869140625]
      mask Display: e = 0.06;c1 = [120 150 230]/255;c2 = ([120 150 230]+0)/383;c3 = ([120 150 230]+128)/383;patch([0 1 1 0],[0 0 1 1],c1);patch([0 1 1 1-e 1-e 0+e],[0 0 1 1-e 0+e 0+e],c2);patch([0 0 1 1-e 0+e 0+e],[0 1 1 1-e 1-e 0+e],c3);plot([0 1 1 0 0],[0 0 1 1 0]);disp('Weights');
  "IW{1,2}(9,:)'" : Constant  Value=[0.0332709230307318970520924494849168695509433746337890625;-0.08712331448893360918983574947560555301606655120849609375;0.0206477017352553367246503768228649278171360492706298828125;-0.1467039621037039276441049651111825369298458099365234375;-0.10458810778853029621604520116306957788765430450439453125;0.0530992277492036979236189608855056576430797576904296875;0.11752914629356514542024569891509599983692169189453125;0.260911515432073415343694477996905334293842315673828125;-0.0286880339646968553213302044468946405686438083648681640625;0.05326019656457785245162739329316536895930767059326171875]
      mask Display: e = 0.06;c1 = [120 150 230]/255;c2 = ([120 150 230]+0)/383;c3 = ([120 150 230]+128)/383;patch([0 1 1 0],[0 0 1 1],c1);patch([0 1 1 1-e 1-e 0+e],[0 0 1 1-e 0+e 0+e],c2);patch([0 0 1 1-e 0+e 0+e],[0 1 1 1-e 1-e 0+e],c3);plot([0 1 1 0 0],[0 0 1 1 0]);disp('Weights');
  "IW{1,2}(90,:)'" : Constant  Value=[-0.00852985907168020938973196365395779139362275600433349609375;-0.0778142996689909771657056580806965939700603485107421875;0.06917121411213666970496660724165849387645721435546875;0.051736083360675255704563824110664427280426025390625;0.0277247832382709231968664909118160721845924854278564453125;0.01433697855228153843210048279388502123765647411346435546875;0.029733760736829116522184079940416268073022365570068359375;-0.029243529646814529765475043632250162772834300994873046875;-0.0020329189846555388403170905320394012960605323314666748046875;-0.0195549509044164147864020009137675515376031398773193359375]
      mask Display: e = 0.06;c1 = [120 150 230]/255;c2 = ([120 150 230]+0)/383;c3 = ([120 150 230]+128)/383;patch([0 1 1 0],[0 0 1 1],c1);patch([0 1 1 1-e 1-e 0+e],[0 0 1 1-e 0+e 0+e],c2);patch([0 0 1 1-e 0+e 0+e],[0 1 1 1-e 1-e 0+e],c3);plot([0 1 1 0 0],[0 0 1 1 0]);disp('Weights');
  "IW{1,2}(91,:)'" : Constant  Value=[-0.007660966851972004186543951931298579438589513301849365234375;-0.07290883707175767336483573899386101402342319488525390625;0.0650626929004527454480921733193099498748779296875;0.048634521201187323746761848042297060601413249969482421875;0.0259042970612273250330392926343847648240625858306884765625;0.0132635871379788439217151108096004463732242584228515625;0.0277977657723960276670016611433311481960117816925048828125;-0.0274718345689367905715361217744430177845060825347900390625;-0.002066469747692918461356992310129498946480453014373779296875;-0.0184651786498333629615853368477473850362002849578857421875]
      mask Display: e = 0.06;c1 = [120 150 230]/255;c2 = ([120 150 230]+0)/383;c3 = ([120 150 230]+128)/383;patch([0 1 1 0],[0 0 1 1],c1);patch([0 1 1 1-e 1-e 0+e],[0 0 1 1-e 0+e 0+e],c2);patch([0 0 1 1-e 0+e 0+e],[0 1 1 1-e 1-e 0+e],c3);plot([0 1 1 0 0],[0 0 1 1 0]);disp('Weights');
  "IW{1,2}(92,:)'" : Constant  Value=[-0.006914483819144110095245014946385708753950893878936767578125;-0.0679041293861308570267709683321299962699413299560546875;0.061222217149560449744871704069737461395561695098876953125;0.04583679154723625803757869334731367416679859161376953125;0.02452451932145187363243366007736767642199993133544921875;0.01265719615639446064825346383031501318328082561492919921875;0.0262796600983170314247416854414041154086589813232421875;-0.02539267984213956774741660638028406538069248199462890625;-0.00165537548197796919972890616890026649343781173229217529296875;-0.0170215619104816147377778889904220704920589923858642578125]
      mask Display: e = 0.06;c1 = [120 150 230]/255;c2 = ([120 150 230]+0)/383;c3 = ([120 150 230]+128)/383;patch([0 1 1 0],[0 0 1 1],c1);patch([0 1 1 1-e 1-e 0+e],[0 0 1 1-e 0+e 0+e],c2);patch([0 0 1 1-e 0+e 0+e],[0 1 1 1-e 1-e 0+e],c3);plot([0 1 1 0 0],[0 0 1 1 0]);disp('Weights');
  "IW{1,2}(93,:)'" : Constant  Value=[-0.1421604347916935184858999718926497735083103179931640625;0.158141245331301527610179391558631323277950286865234375;0.120424830574233643343262656344450078904628753662109375;0.6688246853793915480679288521059788763523101806640625;-0.262580063869036928192457480690791271626949310302734375;-0.1459419049656195677133752042209380306303501129150390625;0.319723110346513517132649440100067295134067535400390625;0.50086099603916089950672585473512299358844757080078125;0.30834270572834887591540109497145749628543853759765625;0.0914204615970774792099717842575046233832836151123046875]
      mask Display: e = 0.06;c1 = [120 150 230]/255;c2 = ([120 150 230]+0)/383;c3 = ([120 150 230]+128)/383;patch([0 1 1 0],[0 0 1 1],c1);patch([0 1 1 1-e 1-e 0+e],[0 0 1 1-e 0+e 0+e],c2);patch([0 0 1 1-e 0+e 0+e],[0 1 1 1-e 1-e 0+e],c3);plot([0 1 1 0 0],[0 0 1 1 0]);disp('Weights');
  "IW{1,2}(94,:)'" : Constant  Value=[0.0078043847294977410078420376748908893205225467681884765625;0.073856004981981637769195003784261643886566162109375;-0.06580325272334690278608348990019294433295726776123046875;-0.04917755679302258930984947937758988700807094573974609375;-0.0261814715718494232798985166255079093389213085174560546875;-0.0133952018509464372553185995684543740935623645782470703125;-0.0281014545730104668697091341300620115362107753753662109375;0.0278567099952216866431964348294059163890779018402099609375;0.0021296046998805022963663358126495950273238122463226318359375;0.01872748197235095390933423686874448321759700775146484375]
      mask Display: e = 0.06;c1 = [120 150 230]/255;c2 = ([120 150 230]+0)/383;c3 = ([120 150 230]+128)/383;patch([0 1 1 0],[0 0 1 1],c1);patch([0 1 1 1-e 1-e 0+e],[0 0 1 1-e 0+e 0+e],c2);patch([0 0 1 1-e 0+e 0+e],[0 1 1 1-e 1-e 0+e],c3);plot([0 1 1 0 0],[0 0 1 1 0]);disp('Weights');
  "IW{1,2}(95,:)'" : Constant  Value=[0.00649080914771942886487554602581440121866762638092041015625;0.06502656976642103014984996889324975199997425079345703125;-0.059028111363531234057067109688432537950575351715087890625;-0.044240446007236540471030394883200642652809619903564453125;-0.0237503909485331059225909910992413642816245555877685546875;-0.012330089627426044085467538025113753974437713623046875;-0.0254256337423934310193462948745946050621569156646728515625;0.0241872732472441613615909972168083186261355876922607421875;0.0014014370582542214939414382257609759108163416385650634765625;0.016179639261357701973675915496642119251191616058349609375]
      mask Display: e = 0.06;c1 = [120 150 230]/255;c2 = ([120 150 230]+0)/383;c3 = ([120 150 230]+128)/383;patch([0 1 1 0],[0 0 1 1],c1);patch([0 1 1 1-e 1-e 0+e],[0 0 1 1-e 0+e 0+e],c2);patch([0 0 1 1-e 0+e 0+e],[0 1 1 1-e 1-e 0+e],c3);plot([0 1 1 0 0],[0 0 1 1 0]);disp('Weights');
  "IW{1,2}(96,:)'" : Constant  Value=[-0.00666737191362338534050824279120206483639776706695556640625;-0.066228582042797967677216774973203428089618682861328125;0.059944670714811292000501197207995573990046977996826171875;0.044907453252490160677812269796049804426729679107666015625;0.024073390070045698474476836281610303558409214019775390625;0.0124661829154301163902207605360672459937632083892822265625;0.0257821271935251596085780789735508733429014682769775390625;-0.0246909286749310181996452939756636624224483966827392578125;-0.0015078367018071148382418744660071752150543034076690673828125;-0.016531449272523916771415741777673247270286083221435546875]
      mask Display: e = 0.06;c1 = [120 150 230]/255;c2 = ([120 150 230]+0)/383;c3 = ([120 150 230]+128)/383;patch([0 1 1 0],[0 0 1 1],c1);patch([0 1 1 1-e 1-e 0+e],[0 0 1 1-e 0+e 0+e],c2);patch([0 0 1 1-e 0+e 0+e],[0 1 1 1-e 1-e 0+e],c3);plot([0 1 1 0 0],[0 0 1 1 0]);disp('Weights');
  "IW{1,2}(97,:)'" : Constant  Value=[-0.0086411293501277471051924550238254596479237079620361328125;-0.07817286736486993292682967648943304084241390228271484375;0.0695155231439378573643494974021450616419315338134765625;0.052013191334096701978761956297603319399058818817138671875;0.02794306390518284943791371688348590396344661712646484375;0.01450074266368374907576477284010252333246171474456787109375;0.029946600514863676301136052870788262225687503814697265625;-0.029319574812132577490420004551197052933275699615478515625;-0.00194686354917464007376060042275867090211249887943267822265625;-0.0195735007225367636796153902878359076566994190216064453125]
      mask Display: e = 0.06;c1 = [120 150 230]/255;c2 = ([120 150 230]+0)/383;c3 = ([120 150 230]+128)/383;patch([0 1 1 0],[0 0 1 1],c1);patch([0 1 1 1-e 1-e 0+e],[0 0 1 1-e 0+e 0+e],c2);patch([0 0 1 1-e 0+e 0+e],[0 1 1 1-e 1-e 0+e],c3);plot([0 1 1 0 0],[0 0 1 1 0]);disp('Weights');
  "IW{1,2}(98,:)'" : Constant  Value=[-0.00695079451014951436860211941848319838754832744598388671875;-0.068149627700214987502391750240349210798740386962890625;0.06140948499656333214868908498829114250838756561279296875;0.045973002202141323435657938034637481905519962310791015625;0.024590797159129686166867401198032894171774387359619140625;0.0126854059549493768110917102376333787105977535247802734375;0.0263527167775604691246638111579159158281981945037841796875;-0.02549541367108525136142560540974955074489116668701171875;-0.00167682977529691923553045729278210274060256779193878173828125;-0.017093280247149005013351796833376283757388591766357421875]
      mask Display: e = 0.06;c1 = [120 150 230]/255;c2 = ([120 150 230]+0)/383;c3 = ([120 150 230]+128)/383;patch([0 1 1 0],[0 0 1 1],c1);patch([0 1 1 1-e 1-e 0+e],[0 0 1 1-e 0+e 0+e],c2);patch([0 0 1 1-e 0+e 0+e],[0 1 1 1-e 1-e 0+e],c3);plot([0 1 1 0 0],[0 0 1 1 0]);disp('Weights');
  "IW{1,2}(99,:)'" : Constant  Value=[-0.30638129570370031817816425245837308466434478759765625;-0.142085445335057125593181126532726921141147613525390625;0.253249031569512172978875241824425756931304931640625;0.415816850395610171364779716896009631454944610595703125;0.38725035820180353507424797498970292508602142333984375;-0.0808705380774039361835292538671637885272502899169921875;0.1096502457501113969584594087791629135608673095703125;-0.10649969655992573558389580057337298057973384857177734375;-0.085110325647811346794213704924914054572582244873046875;-0.03725908744960200469353850394327309913933277130126953125]
      mask Display: e = 0.06;c1 = [120 150 230]/255;c2 = ([120 150 230]+0)/383;c3 = ([120 150 230]+128)/383;patch([0 1 1 0],[0 0 1 1],c1);patch([0 1 1 1-e 1-e 0+e],[0 0 1 1-e 0+e 0+e],c2);patch([0 0 1 1-e 0+e 0+e],[0 1 1 1-e 1-e 0+e],c3);plot([0 1 1 0 0],[0 0 1 1 0]);disp('Weights');
  Mux : Mux  Inputs=100
      mask Display: e = 0.06;c1 = [120 150 230]/255;c2 = ([120 150 230]+0)/383;c3 = ([120 150 230]+128)/383;patch([0 1 1 0],[0 0 1 1],c1);patch([0 1 1 1-e 1-e 0+e],[0 0 1 1-e 0+e 0+e],c2);patch([0 0 1 1-e 0+e 0+e],[0 1 1 1-e 1-e 0+e],c3);plot([0 1 1 0 0],[0 0 1 1 0]);disp('Mux');
  dotprod{1..100} (100 alike) : neural/Weight Functions/dotprod
  "iz{1,2}" : Outport
      mask Display: e = 0.06;c1 = [120 230 180]/255;c2 = ([120 230 180]+0)/(256+128);c3 = ([120 230 180]+128)/(256+128);patch([0 1 1 0],[0 0 1 1],c1);patch([0 1 1 1-e 1-e 0+e],[0 0 1 1-e 0+e 0+e],c2);patch([0 0 1 1-e 0+e 0+e],[0 1 1 1-e 1-e 0+e],c3);plot([0 1 1 0 0],[0 0 1 1 0]);
  wires:
  "IW{1,2}(1,:)'"/1 -> dotprod1/1
  "pd{1,2}"/1 -> dotprod1/2, dotprod2/2, dotprod3/2, dotprod4/2, dotprod5/2, dotprod6/2, dotprod7/2, dotprod8/2, dotprod9/2, dotprod10/2, dotprod11/2, dotprod12/2, dotprod13/2, dotprod14/2, dotprod15/2, dotprod16/2, dotprod17/2, dotprod18/2, dotprod19/2, dotprod20/2, dotprod21/2, dotprod22/2, dotprod23/2, dotprod24/2, dotprod25/2, dotprod26/2, dotprod27/2, dotprod28/2, dotprod29/2, dotprod30/2, dotprod31/2, dotprod32/2, dotprod33/2, dotprod34/2, dotprod35/2, dotprod36/2, dotprod37/2, dotprod38/2, dotprod39/2, dotprod40/2, dotprod41/2, dotprod42/2, dotprod43/2, dotprod44/2, dotprod45/2, dotprod46/2, dotprod47/2, dotprod48/2, dotprod49/2, dotprod50/2, dotprod51/2, dotprod52/2, dotprod53/2, dotprod54/2, dotprod55/2, dotprod56/2, dotprod57/2, dotprod58/2, dotprod59/2, dotprod60/2, dotprod61/2, dotprod62/2, dotprod63/2, dotprod64/2, dotprod65/2, dotprod66/2, dotprod67/2, dotprod68/2, dotprod69/2, dotprod70/2, dotprod71/2, dotprod72/2, dotprod73/2, dotprod74/2, dotprod75/2, dotprod76/2, dotprod77/2, dotprod78/2, dotprod79/2, dotprod80/2, dotprod81/2, dotprod82/2, dotprod83/2, dotprod84/2, dotprod85/2, dotprod86/2, dotprod87/2, dotprod88/2, dotprod89/2, dotprod90/2, dotprod91/2, dotprod92/2, dotprod93/2, dotprod94/2, dotprod95/2, dotprod96/2, dotprod97/2, dotprod98/2, dotprod99/2, dotprod100/2
  dotprod1/1 -> Mux/1
  "IW{1,2}(2,:)'"/1 -> dotprod2/1
  dotprod2/1 -> Mux/2
  "IW{1,2}(3,:)'"/1 -> dotprod3/1
  dotprod3/1 -> Mux/3
  "IW{1,2}(4,:)'"/1 -> dotprod4/1
  dotprod4/1 -> Mux/4
  "IW{1,2}(5,:)'"/1 -> dotprod5/1
  dotprod5/1 -> Mux/5
  "IW{1,2}(6,:)'"/1 -> dotprod6/1
  dotprod6/1 -> Mux/6
  "IW{1,2}(7,:)'"/1 -> dotprod7/1
  dotprod7/1 -> Mux/7
  "IW{1,2}(8,:)'"/1 -> dotprod8/1
  dotprod8/1 -> Mux/8
  "IW{1,2}(9,:)'"/1 -> dotprod9/1
  dotprod9/1 -> Mux/9
  "IW{1,2}(10,:)'"/1 -> dotprod10/1
  dotprod10/1 -> Mux/10
  "IW{1,2}(11,:)'"/1 -> dotprod11/1
  dotprod11/1 -> Mux/11
  "IW{1,2}(12,:)'"/1 -> dotprod12/1
  dotprod12/1 -> Mux/12
  "IW{1,2}(13,:)'"/1 -> dotprod13/1
  dotprod13/1 -> Mux/13
  "IW{1,2}(14,:)'"/1 -> dotprod14/1
  dotprod14/1 -> Mux/14
  "IW{1,2}(15,:)'"/1 -> dotprod15/1
  dotprod15/1 -> Mux/15
  "IW{1,2}(16,:)'"/1 -> dotprod16/1
  dotprod16/1 -> Mux/16
  "IW{1,2}(17,:)'"/1 -> dotprod17/1
  dotprod17/1 -> Mux/17
  "IW{1,2}(18,:)'"/1 -> dotprod18/1
  dotprod18/1 -> Mux/18
  "IW{1,2}(19,:)'"/1 -> dotprod19/1
  dotprod19/1 -> Mux/19
  "IW{1,2}(20,:)'"/1 -> dotprod20/1
  dotprod20/1 -> Mux/20
  "IW{1,2}(21,:)'"/1 -> dotprod21/1
  dotprod21/1 -> Mux/21
  "IW{1,2}(22,:)'"/1 -> dotprod22/1
  dotprod22/1 -> Mux/22
  "IW{1,2}(23,:)'"/1 -> dotprod23/1
  dotprod23/1 -> Mux/23
  "IW{1,2}(24,:)'"/1 -> dotprod24/1
  dotprod24/1 -> Mux/24
  "IW{1,2}(25,:)'"/1 -> dotprod25/1
  dotprod25/1 -> Mux/25
  "IW{1,2}(26,:)'"/1 -> dotprod26/1
  dotprod26/1 -> Mux/26
  "IW{1,2}(27,:)'"/1 -> dotprod27/1
  dotprod27/1 -> Mux/27
  "IW{1,2}(28,:)'"/1 -> dotprod28/1
  dotprod28/1 -> Mux/28
  "IW{1,2}(29,:)'"/1 -> dotprod29/1
  dotprod29/1 -> Mux/29
  "IW{1,2}(30,:)'"/1 -> dotprod30/1
  dotprod30/1 -> Mux/30
  "IW{1,2}(31,:)'"/1 -> dotprod31/1
  dotprod31/1 -> Mux/31
  "IW{1,2}(32,:)'"/1 -> dotprod32/1
  dotprod32/1 -> Mux/32
  "IW{1,2}(33,:)'"/1 -> dotprod33/1
  dotprod33/1 -> Mux/33
  "IW{1,2}(34,:)'"/1 -> dotprod34/1
  dotprod34/1 -> Mux/34
  "IW{1,2}(35,:)'"/1 -> dotprod35/1
  dotprod35/1 -> Mux/35
  "IW{1,2}(36,:)'"/1 -> dotprod36/1
  dotprod36/1 -> Mux/36
  "IW{1,2}(37,:)'"/1 -> dotprod37/1
  dotprod37/1 -> Mux/37
  "IW{1,2}(38,:)'"/1 -> dotprod38/1
  dotprod38/1 -> Mux/38
  "IW{1,2}(39,:)'"/1 -> dotprod39/1
  dotprod39/1 -> Mux/39
  "IW{1,2}(40,:)'"/1 -> dotprod40/1
  dotprod40/1 -> Mux/40
  "IW{1,2}(41,:)'"/1 -> dotprod41/1
  dotprod41/1 -> Mux/41
  "IW{1,2}(42,:)'"/1 -> dotprod42/1
  dotprod42/1 -> Mux/42
  "IW{1,2}(43,:)'"/1 -> dotprod43/1
  dotprod43/1 -> Mux/43
  "IW{1,2}(44,:)'"/1 -> dotprod44/1
  dotprod44/1 -> Mux/44
  "IW{1,2}(45,:)'"/1 -> dotprod45/1
  dotprod45/1 -> Mux/45
  "IW{1,2}(46,:)'"/1 -> dotprod46/1
  dotprod46/1 -> Mux/46
  "IW{1,2}(47,:)'"/1 -> dotprod47/1
  dotprod47/1 -> Mux/47
  "IW{1,2}(48,:)'"/1 -> dotprod48/1
  dotprod48/1 -> Mux/48
  "IW{1,2}(49,:)'"/1 -> dotprod49/1
  dotprod49/1 -> Mux/49
  "IW{1,2}(50,:)'"/1 -> dotprod50/1
  dotprod50/1 -> Mux/50
  "IW{1,2}(51,:)'"/1 -> dotprod51/1
  dotprod51/1 -> Mux/51
  "IW{1,2}(52,:)'"/1 -> dotprod52/1
  dotprod52/1 -> Mux/52
  "IW{1,2}(53,:)'"/1 -> dotprod53/1
  dotprod53/1 -> Mux/53
  "IW{1,2}(54,:)'"/1 -> dotprod54/1
  dotprod54/1 -> Mux/54
  "IW{1,2}(55,:)'"/1 -> dotprod55/1
  dotprod55/1 -> Mux/55
  "IW{1,2}(56,:)'"/1 -> dotprod56/1
  dotprod56/1 -> Mux/56
  "IW{1,2}(57,:)'"/1 -> dotprod57/1
  dotprod57/1 -> Mux/57
  "IW{1,2}(58,:)'"/1 -> dotprod58/1
  dotprod58/1 -> Mux/58
  "IW{1,2}(59,:)'"/1 -> dotprod59/1
  dotprod59/1 -> Mux/59
  "IW{1,2}(60,:)'"/1 -> dotprod60/1
  dotprod60/1 -> Mux/60
  "IW{1,2}(61,:)'"/1 -> dotprod61/1
  dotprod61/1 -> Mux/61
  "IW{1,2}(62,:)'"/1 -> dotprod62/1
  dotprod62/1 -> Mux/62
  "IW{1,2}(63,:)'"/1 -> dotprod63/1
  dotprod63/1 -> Mux/63
  "IW{1,2}(64,:)'"/1 -> dotprod64/1
  dotprod64/1 -> Mux/64
  "IW{1,2}(65,:)'"/1 -> dotprod65/1
  dotprod65/1 -> Mux/65
  "IW{1,2}(66,:)'"/1 -> dotprod66/1
  dotprod66/1 -> Mux/66
  "IW{1,2}(67,:)'"/1 -> dotprod67/1
  dotprod67/1 -> Mux/67
  "IW{1,2}(68,:)'"/1 -> dotprod68/1
  dotprod68/1 -> Mux/68
  "IW{1,2}(69,:)'"/1 -> dotprod69/1
  dotprod69/1 -> Mux/69
  "IW{1,2}(70,:)'"/1 -> dotprod70/1
  dotprod70/1 -> Mux/70
  "IW{1,2}(71,:)'"/1 -> dotprod71/1
  dotprod71/1 -> Mux/71
  "IW{1,2}(72,:)'"/1 -> dotprod72/1
  dotprod72/1 -> Mux/72
  "IW{1,2}(73,:)'"/1 -> dotprod73/1
  dotprod73/1 -> Mux/73
  "IW{1,2}(74,:)'"/1 -> dotprod74/1
  dotprod74/1 -> Mux/74
  "IW{1,2}(75,:)'"/1 -> dotprod75/1
  dotprod75/1 -> Mux/75
  "IW{1,2}(76,:)'"/1 -> dotprod76/1
  dotprod76/1 -> Mux/76
  "IW{1,2}(77,:)'"/1 -> dotprod77/1
  dotprod77/1 -> Mux/77
  "IW{1,2}(78,:)'"/1 -> dotprod78/1
  dotprod78/1 -> Mux/78
  "IW{1,2}(79,:)'"/1 -> dotprod79/1
  dotprod79/1 -> Mux/79
  "IW{1,2}(80,:)'"/1 -> dotprod80/1
  dotprod80/1 -> Mux/80
  "IW{1,2}(81,:)'"/1 -> dotprod81/1
  dotprod81/1 -> Mux/81
  "IW{1,2}(82,:)'"/1 -> dotprod82/1
  dotprod82/1 -> Mux/82
  "IW{1,2}(83,:)'"/1 -> dotprod83/1
  dotprod83/1 -> Mux/83
  "IW{1,2}(84,:)'"/1 -> dotprod84/1
  dotprod84/1 -> Mux/84
  "IW{1,2}(85,:)'"/1 -> dotprod85/1
  dotprod85/1 -> Mux/85
  "IW{1,2}(86,:)'"/1 -> dotprod86/1
  dotprod86/1 -> Mux/86
  "IW{1,2}(87,:)'"/1 -> dotprod87/1
  dotprod87/1 -> Mux/87
  "IW{1,2}(88,:)'"/1 -> dotprod88/1
  dotprod88/1 -> Mux/88
  "IW{1,2}(89,:)'"/1 -> dotprod89/1
  dotprod89/1 -> Mux/89
  "IW{1,2}(90,:)'"/1 -> dotprod90/1
  dotprod90/1 -> Mux/90
  "IW{1,2}(91,:)'"/1 -> dotprod91/1
  dotprod91/1 -> Mux/91
  "IW{1,2}(92,:)'"/1 -> dotprod92/1
  dotprod92/1 -> Mux/92
  "IW{1,2}(93,:)'"/1 -> dotprod93/1
  dotprod93/1 -> Mux/93
  "IW{1,2}(94,:)'"/1 -> dotprod94/1
  dotprod94/1 -> Mux/94
  "IW{1,2}(95,:)'"/1 -> dotprod95/1
  dotprod95/1 -> Mux/95
  "IW{1,2}(96,:)'"/1 -> dotprod96/1
  dotprod96/1 -> Mux/96
  "IW{1,2}(97,:)'"/1 -> dotprod97/1
  dotprod97/1 -> Mux/97
  "IW{1,2}(98,:)'"/1 -> dotprod98/1
  dotprod98/1 -> Mux/98
  "IW{1,2}(99,:)'"/1 -> dotprod99/1
  dotprod99/1 -> Mux/99
  "IW{1,2}(100,:)'"/1 -> dotprod100/1
  dotprod100/1 -> Mux/100
  Mux/1 -> "iz{1,2}"/1
